simulink model "CRTsfun"  (Simulink 8.0)
settings: Solver=ode45  StartTime=0.0  StopTime=10.0  RelTol=1e-3
undefined symbols (not defined in the file or in its folder): vicrt_initcallback, vicrt_initmexcallback, vicrt_inputfile, vicrt_simulationmanager
(part 2 of 3)

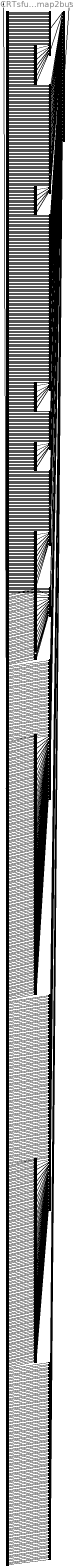
== system CRTsfun/VI-CarRealTime/Output_Bus/IOmap2bus ==
  In : Inport
  Actual_Tread_Speed : BusCreator
  Aggregate_Force_At_Wheel : BusCreator
  Alpha : BusCreator
  Animator_Widget : BusCreator  Inputs=2
  Auxiliary_Roll_Force : BusCreator
  Auxiliary_Roll_Force_at_element : BusCreator  Inputs=2
  Auxiliary_Roll_deformation_at_element : BusCreator  Inputs=2
  Brake : BusCreator  Inputs=7
  Brake_Moment : BusCreator
  Caster_Angle : BusCreator  Inputs=2
  Chamber_Pressure : BusCreator
  Contact_Patch_Global_X : BusCreator
  Contact_Patch_Global_Y : BusCreator
  Contact_Patch_Global_Z : BusCreator
  Contact_Patch_Global_dZdX : BusCreator
  Contact_Patch_Global_dZdY : BusCreator
  Damper : BusCreator  Inputs=5
  Demux : Demux  Outputs=1100
  Drive_Moment : BusCreator
  Effective_Closing_Speed : BusCreator
  Effective_Penetration : BusCreator
  Effective_Rolling_Radius : BusCreator
  Equivalent_Tread_Speed : BusCreator
  Euler_Roll : BusCreator
  External_Friction_Scale_Factor : BusCreator
  Force_At_Bumper : BusCreator
  Force_At_Bumper1 : BusCreator
  Force_At_Damper : BusCreator
  Force_At_Spring : BusCreator
  Force_At_Wheel{,1..3} (4 alike) : BusCreator
  Force_Aux_At_Wheel : BusCreator
  Global_Omega_X : BusCreator
  Global_Omega_Y : BusCreator
  Global_Omega_Z : BusCreator
  Global_Vx : BusCreator
  Global_Vy : BusCreator
  Global_Vz : BusCreator
  Global_X : BusCreator
  Global_Y : BusCreator
  Global_Z : BusCreator
  Ground_Surface_Contact_Patch_Vx : BusCreator
  Ground_Surface_Contact_Patch_Vy : BusCreator
  Ground_Surface_Force_X : BusCreator
  Ground_Surface_Force_Y : BusCreator
  Ground_Surface_Force_Z : BusCreator
  Ground_Surface_Gyroscopic_Moment : BusCreator
  Ground_Surface_Kappa_Fy : BusCreator
  Ground_Surface_Moment_X : BusCreator
  Ground_Surface_Moment_Y : BusCreator
  Ground_Surface_Moment_Z : BusCreator
  Ground_Surface_Peak_Friction_X : BusCreator
  Ground_Surface_Peak_Friction_Y : BusCreator
  Ground_Surface_Residual_Torque : BusCreator
  Ground_Surface_Wheel_Center_Vx : BusCreator
  Gyro : BusCreator  Inputs=10
  Hook_rear : BusCreator  Inputs=18
  Hub_Carrier_Force_Global_X : BusCreator
  Hub_Carrier_Force_Global_Y : BusCreator
  Hub_Carrier_Force_Global_Z : BusCreator
  Hub_Carrier_Force_Local_X : BusCreator
  Hub_Carrier_Force_Local_Y : BusCreator
  Hub_Carrier_Force_Local_Z : BusCreator
  Hub_Carrier_Moment_Global_X : BusCreator
  Hub_Carrier_Moment_Global_Y : BusCreator
  Hub_Carrier_Moment_Global_Z : BusCreator
  Hub_Carrier_Moment_Local_X : BusCreator
  Hub_Carrier_Moment_Local_Y : BusCreator
  Hub_Carrier_Moment_Local_Z : BusCreator
  Hub_Carrier_Omega_X : BusCreator
  Hub_Carrier_Omega_Y : BusCreator
  Hub_Carrier_Omega_Z : BusCreator
  Hub_Carrier_Vx : BusCreator
  Hub_Carrier_Vy : BusCreator
  Hub_Carrier_Vz : BusCreator
  Inclination : BusCreator
  Inst_Stiff_Deflection : BusCreator
  Inst_Stiff_Force : BusCreator
  Jounce{,1..4} (5 alike) : BusCreator
  Jounce_Acceleration{,1..4} (5 alike) : BusCreator
  Jounce_Bumper : BusCreator  Inputs=5
  Jounce_Rate{,1..4} (5 alike) : BusCreator
  Kingpin_Moment : BusCreator  Inputs=1
  Kingpin_Moment1 : BusCreator  Inputs=2
  Lateral_Relaxation_Length : BusCreator
  Lateral_Slip_With_Lag : BusCreator
  Lateral_Slip_Without_Lag : BusCreator
  Loaded_Radius : BusCreator
  Locked_Damper_Moment : BusCreator
  Locked_Moment : BusCreator
  Locked_Spring_Moment : BusCreator
  Locked_Switch : BusCreator
  Lockup_Rotation : BusCreator
  Longitudinal_Relaxation_Length : BusCreator
  Longitudinal_Slip_With_Lag : BusCreator
  Longitudinal_Slip_Without_Lag : BusCreator
  Moment_Arm_Of_Fx : BusCreator
  Omega : BusCreator
  OutputBus : BusCreator  Inputs=92
  PID_CW_At_Spring : BusCreator
  PID_PH_At_Spring : BusCreator
  PID_RH_At_Spring : BusCreator
  Phi : BusCreator
  Pitch : BusCreator
  Pneumatic_Trail : BusCreator
  Psi : BusCreator
  Rebound_Bumper : BusCreator  Inputs=5
  Roll : BusCreator  Inputs=2
  Rotation : BusCreator
  Sensor : BusCreator  Inputs=16
  Side_View_Angle : BusCreator
  Spindle_Steer : BusCreator
  Spring : BusCreator  Inputs=10
  Steering_Instant_Axis_Rotation : BusCreator  Inputs=2
  Steering_System : BusCreator  Inputs=6
  Suspension : BusCreator  Inputs=14
  System : BusCreator
  System_Mass_Center : BusCreator  Inputs=13
  Theta : BusCreator
  TieRod_Force_Left : BusCreator  Inputs=3
  TieRod_Force_Right : BusCreator  Inputs=3
  Tire : BusCreator  Inputs=46
  User_Input_Contact_Patch_Global_Z_Perturbation : BusCreator
  Vehicle : BusCreator  Inputs=46
  Vehicle_States : BusCreator  Inputs=20
  Wheel : BusCreator  Inputs=37
  Yaw : BusCreator
  aero_forces : BusCreator  Inputs=24
  base_acceleration : BusCreator
  base_deformation : BusCreator
  base_velocity : BusCreator
  bul_jounce_stop_data : BusCreator
  bul_rebound_stop_data : BusCreator
  bur_jounce_stop_data : BusCreator
  bur_rebound_stop_data : BusCreator
  bus_dmp_jounce_stop_data : BusCreator  Inputs=6
  bus_ins_jounce_stop_data : BusCreator  Inputs=6
  bus_roll_dmp_jounce_stop_data : BusCreator  Inputs=6
  bus_spr_jounce_stop_data : BusCreator  Inputs=6
  chassis_accelerations : BusCreator  Inputs=6
  chassis_displacements : BusCreator  Inputs=9
  chassis_velocities : BusCreator  Inputs=6
  clutch : BusCreator  Inputs=2
  condition_sensors : BusCreator  Inputs=1
  cp_force_lateralFL : BusCreator  Inputs=3
  cp_force_lateralFR : BusCreator  Inputs=3
  cp_force_lateralRL : BusCreator  Inputs=3
  cp_force_lateralRR : BusCreator  Inputs=3
  cp_force_longitudinalFL : BusCreator  Inputs=3
  cp_force_longitudinalFR : BusCreator  Inputs=3
  cp_force_longitudinalRL : BusCreator  Inputs=3
  cp_force_longitudinalRR : BusCreator  Inputs=3
  cp_force_normalFL : BusCreator  Inputs=3
  cp_force_normalFR : BusCreator  Inputs=3
  cp_force_normalRL : BusCreator  Inputs=3
  cp_force_normalRR : BusCreator  Inputs=3
  cross_weight : BusCreator
  dal_ride_damper_data : BusCreator
  dar_ride_damper_data : BusCreator
  das_ride_damper_data : BusCreator  Inputs=6
  das_roll_damper_data : BusCreator  Inputs=8
  das_third_damper_data : BusCreator  Inputs=6
  differential_speeds : BusCreator  Inputs=6
  differential_torques : BusCreator  Inputs=6
  driver_demands : BusCreator  Inputs=7
  driving_machine_monitor : BusCreator  Inputs=9
  engine : BusCreator  Inputs=7
  fuel_consumption : BusCreator
  ges_chassis_XFORM : BusCreator  Inputs=6
  ges_hub_XFORMFL : BusCreator  Inputs=6
  ges_hub_XFORMFR : BusCreator  Inputs=6
  ges_hub_XFORMRL : BusCreator  Inputs=6
  ges_hub_XFORMRR : BusCreator  Inputs=6
  hub2cp_XFORMFL : BusCreator  Inputs=3
  hub2cp_XFORMFR : BusCreator  Inputs=3
  hub2cp_XFORMRL : BusCreator  Inputs=3
  hub2cp_XFORMRR : BusCreator  Inputs=3
  hub_center_accx : BusCreator
  hub_center_accy : BusCreator
  hub_center_accz : BusCreator
  ins_inerter_data : BusCreator  Inputs=10
  jfs_torsional_stiffness_data : BusCreator  Inputs=12
  nsl_ride_spring_data : BusCreator  Inputs=6
  nsr_ride_spring_data : BusCreator  Inputs=6
  nss_ride_spring_data : BusCreator  Inputs=10
  res_dmp_rebound_stop_data : BusCreator  Inputs=6
  res_ins_rebound_stop_data : BusCreator  Inputs=6
  res_roll_dmp_rebound_stop_data : BusCreator  Inputs=6
  res_spr_rebound_stop_data : BusCreator  Inputs=6
  rhl_front_setup_sensor_data : BusCreator  Inputs=1
  rhr_front_setup_sensor_data : BusCreator  Inputs=1
  rhs_rear_setup_sensor_data : BusCreator  Inputs=1
  til_wheel_tire_forces : BusCreator  Inputs=18
  til_wheel_tire_kinematics : BusCreator  Inputs=9
  til_wheel_tire_rolling_states : BusCreator  Inputs=9
  tir_wheel_tire_forces : BusCreator  Inputs=18
  tir_wheel_tire_kinematics : BusCreator  Inputs=9
  tir_wheel_tire_rolling_states : BusCreator  Inputs=9
  transmission : BusCreator
  ues_third_spring_data : BusCreator  Inputs=6
  upright_accelerometer : BusCreator
  wheel_angles : BusCreator  Inputs=12
  wheel_center_dispx : BusCreator
  wheel_center_dispy : BusCreator
  wheel_center_dispz : BusCreator
  whl_front_wheel_XFORM : BusCreator  Inputs=9
  whl_rear_wheel_XFORM : BusCreator  Inputs=9
  whl_twin_rear_wheel_XFORM : BusCreator  Inputs=9
  whr_front_wheel_XFORM : BusCreator  Inputs=9
  whr_rear_wheel_XFORM : BusCreator  Inputs=9
  whr_twin_rear_wheel_XFORM : BusCreator  Inputs=9
  Out : Outport
  wires:
  Demux/1100 -> cp_force_normalRR/3  "Z"
  Demux/1099 -> cp_force_normalRR/2  "Y"
  Demux/1098 -> cp_force_normalRR/1  "X"
  cp_force_normalRR/1 -> OutputBus/92  "cp_force_normalRR"
  Demux/1097 -> cp_force_lateralRR/3  "Z"
  Demux/1096 -> cp_force_lateralRR/2  "Y"
  Demux/1095 -> cp_force_lateralRR/1  "X"
  cp_force_lateralRR/1 -> OutputBus/91  "cp_force_lateralRR"
  Demux/1094 -> cp_force_longitudinalRR/3  "Z"
  Demux/1093 -> cp_force_longitudinalRR/2  "Y"
  Demux/1092 -> cp_force_longitudinalRR/1  "X"
  cp_force_longitudinalRR/1 -> OutputBus/90  "cp_force_longitudinalRR"
  Demux/1091 -> hub2cp_XFORMRR/3  "Z"
  Demux/1090 -> hub2cp_XFORMRR/2  "Y"
  Demux/1089 -> hub2cp_XFORMRR/1  "X"
  hub2cp_XFORMRR/1 -> OutputBus/89  "hub2cp_XFORMRR"
  Demux/1088 -> ges_hub_XFORMRR/6  "Phi"
  Demux/1087 -> ges_hub_XFORMRR/5  "Theta"
  Demux/1086 -> ges_hub_XFORMRR/4  "Psi"
  Demux/1085 -> ges_hub_XFORMRR/3  "Z"
  Demux/1084 -> ges_hub_XFORMRR/2  "Y"
  Demux/1083 -> ges_hub_XFORMRR/1  "X"
  ges_hub_XFORMRR/1 -> OutputBus/88  "ges_hub_XFORMRR"
  Demux/1082 -> cp_force_normalRL/3  "Z"
  Demux/1081 -> cp_force_normalRL/2  "Y"
  Demux/1080 -> cp_force_normalRL/1  "X"
  cp_force_normalRL/1 -> OutputBus/87  "cp_force_normalRL"
  Demux/1079 -> cp_force_lateralRL/3  "Z"
  Demux/1078 -> cp_force_lateralRL/2  "Y"
  Demux/1077 -> cp_force_lateralRL/1  "X"
  cp_force_lateralRL/1 -> OutputBus/86  "cp_force_lateralRL"
  Demux/1076 -> cp_force_longitudinalRL/3  "Z"
  Demux/1075 -> cp_force_longitudinalRL/2  "Y"
  Demux/1074 -> cp_force_longitudinalRL/1  "X"
  cp_force_longitudinalRL/1 -> OutputBus/85  "cp_force_longitudinalRL"
  Demux/1073 -> hub2cp_XFORMRL/3  "Z"
  Demux/1072 -> hub2cp_XFORMRL/2  "Y"
  Demux/1071 -> hub2cp_XFORMRL/1  "X"
  hub2cp_XFORMRL/1 -> OutputBus/84  "hub2cp_XFORMRL"
  Demux/1070 -> ges_hub_XFORMRL/6  "Phi"
  Demux/1069 -> ges_hub_XFORMRL/5  "Theta"
  Demux/1068 -> ges_hub_XFORMRL/4  "Psi"
  Demux/1067 -> ges_hub_XFORMRL/3  "Z"
  Demux/1066 -> ges_hub_XFORMRL/2  "Y"
  Demux/1065 -> ges_hub_XFORMRL/1  "X"
  ges_hub_XFORMRL/1 -> OutputBus/83  "ges_hub_XFORMRL"
  Demux/1064 -> cp_force_normalFR/3  "Z"
  Demux/1063 -> cp_force_normalFR/2  "Y"
  Demux/1062 -> cp_force_normalFR/1  "X"
  cp_force_normalFR/1 -> OutputBus/82  "cp_force_normalFR"
  Demux/1061 -> cp_force_lateralFR/3  "Z"
  Demux/1060 -> cp_force_lateralFR/2  "Y"
  Demux/1059 -> cp_force_lateralFR/1  "X"
  cp_force_lateralFR/1 -> OutputBus/81  "cp_force_lateralFR"
  Demux/1058 -> cp_force_longitudinalFR/3  "Z"
  Demux/1057 -> cp_force_longitudinalFR/2  "Y"
  Demux/1056 -> cp_force_longitudinalFR/1  "X"
  cp_force_longitudinalFR/1 -> OutputBus/80  "cp_force_longitudinalFR"
  Demux/1055 -> hub2cp_XFORMFR/3  "Z"
  Demux/1054 -> hub2cp_XFORMFR/2  "Y"
  Demux/1053 -> hub2cp_XFORMFR/1  "X"
  hub2cp_XFORMFR/1 -> OutputBus/79  "hub2cp_XFORMFR"
  Demux/1052 -> ges_hub_XFORMFR/6  "Phi"
  Demux/1051 -> ges_hub_XFORMFR/5  "Theta"
  Demux/1050 -> ges_hub_XFORMFR/4  "Psi"
  Demux/1049 -> ges_hub_XFORMFR/3  "Z"
  Demux/1048 -> ges_hub_XFORMFR/2  "Y"
  Demux/1047 -> ges_hub_XFORMFR/1  "X"
  ges_hub_XFORMFR/1 -> OutputBus/78  "ges_hub_XFORMFR"
  Demux/1046 -> cp_force_normalFL/3  "Z"
  Demux/1045 -> cp_force_normalFL/2  "Y"
  Demux/1044 -> cp_force_normalFL/1  "X"
  cp_force_normalFL/1 -> OutputBus/77  "cp_force_normalFL"
  Demux/1043 -> cp_force_lateralFL/3  "Z"
  Demux/1042 -> cp_force_lateralFL/2  "Y"
  Demux/1041 -> cp_force_lateralFL/1  "X"
  cp_force_lateralFL/1 -> OutputBus/76  "cp_force_lateralFL"
  Demux/1040 -> cp_force_longitudinalFL/3  "Z"
  Demux/1039 -> cp_force_longitudinalFL/2  "Y"
  Demux/1038 -> cp_force_longitudinalFL/1  "X"
  cp_force_longitudinalFL/1 -> OutputBus/75  "cp_force_longitudinalFL"
  Demux/1037 -> hub2cp_XFORMFL/3  "Z"
  Demux/1036 -> hub2cp_XFORMFL/2  "Y"
  Demux/1035 -> hub2cp_XFORMFL/1  "X"
  hub2cp_XFORMFL/1 -> OutputBus/74  "hub2cp_XFORMFL"
  Demux/1034 -> ges_hub_XFORMFL/6  "Phi"
  Demux/1033 -> ges_hub_XFORMFL/5  "Theta"
  Demux/1032 -> ges_hub_XFORMFL/4  "Psi"
  Demux/1031 -> ges_hub_XFORMFL/3  "Z"
  Demux/1030 -> ges_hub_XFORMFL/2  "Y"
  Demux/1029 -> ges_hub_XFORMFL/1  "X"
  ges_hub_XFORMFL/1 -> OutputBus/73  "ges_hub_XFORMFL"
  Demux/1028 -> Animator_Widget/2  "engine_rpm"
  Demux/1027 -> Animator_Widget/1  "longitudinal_speed"
  Animator_Widget/1 -> OutputBus/72  "Animator_Widget"
  Demux/1026 -> whr_twin_rear_wheel_XFORM/9  "Z"
  Demux/1025 -> whr_twin_rear_wheel_XFORM/8  "Y"
  Demux/1024 -> whr_twin_rear_wheel_XFORM/7  "X"
  Demux/1023 -> whr_twin_rear_wheel_XFORM/6  "Theta"
  Demux/1022 -> whr_twin_rear_wheel_XFORM/5  "Psi"
  Demux/1021 -> whr_twin_rear_wheel_XFORM/4  "Phi"
  Demux/1020 -> whr_twin_rear_wheel_XFORM/3  "FZ"
  Demux/1019 -> whr_twin_rear_wheel_XFORM/2  "FY"
  Demux/1018 -> whr_twin_rear_wheel_XFORM/1  "FX"
  whr_twin_rear_wheel_XFORM/1 -> OutputBus/71  "whr_twin_rear_wheel_XFORM"
  Demux/1017 -> whr_rear_wheel_XFORM/9  "Z"
  Demux/1016 -> whr_rear_wheel_XFORM/8  "Y"
  Demux/1015 -> whr_rear_wheel_XFORM/7  "X"
  Demux/1014 -> whr_rear_wheel_XFORM/6  "Theta"
  Demux/1013 -> whr_rear_wheel_XFORM/5  "Psi"
  Demux/1012 -> whr_rear_wheel_XFORM/4  "Phi"
  Demux/1011 -> whr_rear_wheel_XFORM/3  "FZ"
  Demux/1010 -> whr_rear_wheel_XFORM/2  "FY"
  Demux/1009 -> whr_rear_wheel_XFORM/1  "FX"
  whr_rear_wheel_XFORM/1 -> OutputBus/70  "whr_rear_wheel_XFORM"
  Demux/1008 -> whr_front_wheel_XFORM/9  "Z"
  Demux/1007 -> whr_front_wheel_XFORM/8  "Y"
  Demux/1006 -> whr_front_wheel_XFORM/7  "X"
  Demux/1005 -> whr_front_wheel_XFORM/6  "Theta"
  Demux/1004 -> whr_front_wheel_XFORM/5  "Psi"
  Demux/1003 -> whr_front_wheel_XFORM/4  "Phi"
  Demux/1002 -> whr_front_wheel_XFORM/3  "FZ"
  Demux/1001 -> whr_front_wheel_XFORM/2  "FY"
  Demux/1000 -> whr_front_wheel_XFORM/1  "FX"
  whr_front_wheel_XFORM/1 -> OutputBus/69  "whr_front_wheel_XFORM"
  Demux/999 -> whl_twin_rear_wheel_XFORM/9  "Z"
  Demux/998 -> whl_twin_rear_wheel_XFORM/8  "Y"
  Demux/997 -> whl_twin_rear_wheel_XFORM/7  "X"
  Demux/996 -> whl_twin_rear_wheel_XFORM/6  "Theta"
  Demux/995 -> whl_twin_rear_wheel_XFORM/5  "Psi"
  Demux/994 -> whl_twin_rear_wheel_XFORM/4  "Phi"
  Demux/993 -> whl_twin_rear_wheel_XFORM/3  "FZ"
  Demux/992 -> whl_twin_rear_wheel_XFORM/2  "FY"
  Demux/991 -> whl_twin_rear_wheel_XFORM/1  "FX"
  whl_twin_rear_wheel_XFORM/1 -> OutputBus/68  "whl_twin_rear_wheel_XFORM"
  Demux/990 -> whl_rear_wheel_XFORM/9  "Z"
  Demux/989 -> whl_rear_wheel_XFORM/8  "Y"
  Demux/988 -> whl_rear_wheel_XFORM/7  "X"
  Demux/987 -> whl_rear_wheel_XFORM/6  "Theta"
  Demux/986 -> whl_rear_wheel_XFORM/5  "Psi"
  Demux/985 -> whl_rear_wheel_XFORM/4  "Phi"
  Demux/984 -> whl_rear_wheel_XFORM/3  "FZ"
  Demux/983 -> whl_rear_wheel_XFORM/2  "FY"
  Demux/982 -> whl_rear_wheel_XFORM/1  "FX"
  whl_rear_wheel_XFORM/1 -> OutputBus/67  "whl_rear_wheel_XFORM"
  Demux/981 -> whl_front_wheel_XFORM/9  "Z"
  Demux/980 -> whl_front_wheel_XFORM/8  "Y"
  Demux/979 -> whl_front_wheel_XFORM/7  "X"
  Demux/978 -> whl_front_wheel_XFORM/6  "Theta"
  Demux/977 -> whl_front_wheel_XFORM/5  "Psi"
  Demux/976 -> whl_front_wheel_XFORM/4  "Phi"
  Demux/975 -> whl_front_wheel_XFORM/3  "FZ"
  Demux/974 -> whl_front_wheel_XFORM/2  "FY"
  Demux/973 -> whl_front_wheel_XFORM/1  "FX"
  whl_front_wheel_XFORM/1 -> OutputBus/66  "whl_front_wheel_XFORM"
  Demux/972 -> wheel_angles/12  "toe_R2"
  Demux/971 -> wheel_angles/11  "toe_R1"
  Demux/970 -> wheel_angles/10  "toe_L2"
  Demux/969 -> wheel_angles/9  "toe_L1"
  Demux/968 -> wheel_angles/8  "caster_R2"
  Demux/967 -> wheel_angles/7  "caster_R1"
  Demux/966 -> wheel_angles/6  "caster_L2"
  Demux/965 -> wheel_angles/5  "caster_L1"
  Demux/964 -> wheel_angles/4  "camber_R2"
  Demux/963 -> wheel_angles/3  "camber_R1"
  Demux/962 -> wheel_angles/2  "camber_L2"
  Demux/961 -> wheel_angles/1  "camber_L1"
  wheel_angles/1 -> OutputBus/65  "wheel_angles"
  Demux/960 -> Yaw/4  "R2"
  Demux/959 -> Yaw/3  "R1"
  Demux/958 -> Yaw/2  "L2"
  Demux/957 -> Yaw/1  "L1"
  Yaw/1 -> Wheel/37  "Yaw"
  Demux/956 -> wheel_center_dispz/4  "rear_right"
  Demux/955 -> wheel_center_dispz/3  "rear_left"
  Demux/954 -> wheel_center_dispz/2  "front_right"
  Demux/953 -> wheel_center_dispz/1  "front_left"
  wheel_center_dispz/1 -> Wheel/36  "wheel_center_dispz"
  Demux/952 -> wheel_center_dispy/4  "rear_right"
  Demux/951 -> wheel_center_dispy/3  "rear_left"
  Demux/950 -> wheel_center_dispy/2  "front_right"
  Demux/949 -> wheel_center_dispy/1  "front_left"
  wheel_center_dispy/1 -> Wheel/35  "wheel_center_dispy"
  Demux/948 -> wheel_center_dispx/4  "rear_right"
  Demux/947 -> wheel_center_dispx/3  "rear_left"
  Demux/946 -> wheel_center_dispx/2  "front_right"
  Demux/945 -> wheel_center_dispx/1  "front_left"
  wheel_center_dispx/1 -> Wheel/34  "wheel_center_dispx"
  Demux/944 -> Theta/4  "R2"
  Demux/943 -> Theta/3  "R1"
  Demux/942 -> Theta/2  "L2"
  Demux/941 -> Theta/1  "L1"
  Theta/1 -> Wheel/33  "Theta"
  Demux/940 -> Spindle_Steer/4  "R2"
  Demux/939 -> Spindle_Steer/3  "R1"
  Demux/938 -> Spindle_Steer/2  "L2"
  Demux/937 -> Spindle_Steer/1  "L1"
  Spindle_Steer/1 -> Wheel/32  "Spindle_Steer"
  Demux/936 -> Side_View_Angle/4  "R2"
  Demux/935 -> Side_View_Angle/3  "R1"
  Demux/934 -> Side_View_Angle/2  "L2"
  Demux/933 -> Side_View_Angle/1  "L1"
  Side_View_Angle/1 -> Wheel/31  "Side_View_Angle"
  Demux/932 -> Rotation/4  "R2"
  Demux/931 -> Rotation/3  "R1"
  Demux/930 -> Rotation/2  "L2"
  Demux/929 -> Rotation/1  "L1"
  Rotation/1 -> Wheel/30  "Rotation"
  Demux/928 -> Psi/4  "R2"
  Demux/927 -> Psi/3  "R1"
  Demux/926 -> Psi/2  "L2"
  Demux/925 -> Psi/1  "L1"
  Psi/1 -> Wheel/29  "Psi"
  Demux/924 -> Pitch/4  "R2"
  Demux/923 -> Pitch/3  "R1"
  Demux/922 -> Pitch/2  "L2"
  Demux/921 -> Pitch/1  "L1"
  Pitch/1 -> Wheel/28  "Pitch"
  Demux/920 -> Phi/4  "R2"
  Demux/919 -> Phi/3  "R1"
  Demux/918 -> Phi/2  "L2"
  Demux/917 -> Phi/1  "L1"
  Phi/1 -> Wheel/27  "Phi"
  Demux/916 -> Omega/4  "R2"
  Demux/915 -> Omega/3  "R1"
  Demux/914 -> Omega/2  "L2"
  Demux/913 -> Omega/1  "L1"
  Omega/1 -> Wheel/26  "Omega"
  Demux/912 -> Kingpin_Moment1/2  "R1"
  Demux/911 -> Kingpin_Moment1/1  "L1"
  Kingpin_Moment1/1 -> Wheel/25  "Kingpin_Moment"
  Demux/910 -> Inclination/4  "R2"
  Demux/909 -> Inclination/3  "R1"
  Demux/908 -> Inclination/2  "L2"
  Demux/907 -> Inclination/1  "L1"
  Inclination/1 -> Wheel/24  "Inclination"
  Demux/906 -> hub_center_accz/4  "rear_right"
  Demux/905 -> hub_center_accz/3  "rear_left"
  Demux/904 -> hub_center_accz/2  "front_right"
  Demux/903 -> hub_center_accz/1  "front_left"
  hub_center_accz/1 -> Wheel/23  "hub_center_accz"
  Demux/902 -> hub_center_accy/4  "rear_right"
  Demux/901 -> hub_center_accy/3  "rear_left"
  Demux/900 -> hub_center_accy/2  "front_right"
  Demux/899 -> hub_center_accy/1  "front_left"
  hub_center_accy/1 -> Wheel/22  "hub_center_accy"
  Demux/898 -> hub_center_accx/4  "rear_right"
  Demux/897 -> hub_center_accx/3  "rear_left"
  Demux/896 -> hub_center_accx/2  "front_right"
  Demux/895 -> hub_center_accx/1  "front_left"
  hub_center_accx/1 -> Wheel/21  "hub_center_accx"
  Demux/894 -> Hub_Carrier_Vz/4  "R2"
  Demux/893 -> Hub_Carrier_Vz/3  "R1"
  Demux/892 -> Hub_Carrier_Vz/2  "L2"
  Demux/891 -> Hub_Carrier_Vz/1  "L1"
  Hub_Carrier_Vz/1 -> Wheel/20  "Hub_Carrier_Vz"
  Demux/890 -> Hub_Carrier_Vy/4  "R2"
  Demux/889 -> Hub_Carrier_Vy/3  "R1"
  Demux/888 -> Hub_Carrier_Vy/2  "L2"
  Demux/887 -> Hub_Carrier_Vy/1  "L1"
  Hub_Carrier_Vy/1 -> Wheel/19  "Hub_Carrier_Vy"
  Demux/886 -> Hub_Carrier_Vx/4  "R2"
  Demux/885 -> Hub_Carrier_Vx/3  "R1"
  Demux/884 -> Hub_Carrier_Vx/2  "L2"
  Demux/883 -> Hub_Carrier_Vx/1  "L1"
  Hub_Carrier_Vx/1 -> Wheel/18  "Hub_Carrier_Vx"
  Demux/882 -> Hub_Carrier_Omega_Z/4  "R2"
  Demux/881 -> Hub_Carrier_Omega_Z/3  "R1"
  Demux/880 -> Hub_Carrier_Omega_Z/2  "L2"
  Demux/879 -> Hub_Carrier_Omega_Z/1  "L1"
  Hub_Carrier_Omega_Z/1 -> Wheel/17  "Hub_Carrier_Omega_Z"
  Demux/878 -> Hub_Carrier_Omega_Y/4  "R2"
  Demux/877 -> Hub_Carrier_Omega_Y/3  "R1"
  Demux/876 -> Hub_Carrier_Omega_Y/2  "L2"
  Demux/875 -> Hub_Carrier_Omega_Y/1  "L1"
  Hub_Carrier_Omega_Y/1 -> Wheel/16  "Hub_Carrier_Omega_Y"
  Demux/874 -> Hub_Carrier_Omega_X/4  "R2"
  Demux/873 -> Hub_Carrier_Omega_X/3  "R1"
  Demux/872 -> Hub_Carrier_Omega_X/2  "L2"
  Demux/871 -> Hub_Carrier_Omega_X/1  "L1"
  Hub_Carrier_Omega_X/1 -> Wheel/15  "Hub_Carrier_Omega_X"
  Demux/870 -> Ground_Surface_Wheel_Center_Vx/4  "R2"
  Demux/869 -> Ground_Surface_Wheel_Center_Vx/3  "R1"
  Demux/868 -> Ground_Surface_Wheel_Center_Vx/2  "L2"
  Demux/867 -> Ground_Surface_Wheel_Center_Vx/1  "L1"
  Ground_Surface_Wheel_Center_Vx/1 -> Wheel/14  "Ground_Surface_Wheel_Center_Vx"
  Demux/866 -> Global_Z/4  "R2"
  Demux/865 -> Global_Z/3  "R1"
  Demux/864 -> Global_Z/2  "L2"
  Demux/863 -> Global_Z/1  "L1"
  Global_Z/1 -> Wheel/13  "Global_Z"
  Demux/862 -> Global_Y/4  "R2"
  Demux/861 -> Global_Y/3  "R1"
  Demux/860 -> Global_Y/2  "L2"
  Demux/859 -> Global_Y/1  "L1"
  Global_Y/1 -> Wheel/12  "Global_Y"
  Demux/858 -> Global_X/4  "R2"
  Demux/857 -> Global_X/3  "R1"
  Demux/856 -> Global_X/2  "L2"
  Demux/855 -> Global_X/1  "L1"
  Global_X/1 -> Wheel/11  "Global_X"
  Demux/854 -> Global_Vz/4  "R2"
  Demux/853 -> Global_Vz/3  "R1"
  Demux/852 -> Global_Vz/2  "L2"
  Demux/851 -> Global_Vz/1  "L1"
  Global_Vz/1 -> Wheel/10  "Global_Vz"
  Demux/850 -> Global_Vy/4  "R2"
  Demux/849 -> Global_Vy/3  "R1"
  Demux/848 -> Global_Vy/2  "L2"
  Demux/847 -> Global_Vy/1  "L1"
  Global_Vy/1 -> Wheel/9  "Global_Vy"
  Demux/846 -> Global_Vx/4  "R2"
  Demux/845 -> Global_Vx/3  "R1"
  Demux/844 -> Global_Vx/2  "L2"
  Demux/843 -> Global_Vx/1  "L1"
  Global_Vx/1 -> Wheel/8  "Global_Vx"
  Demux/842 -> Global_Omega_Z/4  "R2"
  Demux/841 -> Global_Omega_Z/3  "R1"
  Demux/840 -> Global_Omega_Z/2  "L2"
  Demux/839 -> Global_Omega_Z/1  "L1"
  Global_Omega_Z/1 -> Wheel/7  "Global_Omega_Z"
  Demux/838 -> Global_Omega_Y/4  "R2"
  Demux/837 -> Global_Omega_Y/3  "R1"
  Demux/836 -> Global_Omega_Y/2  "L2"
  Demux/835 -> Global_Omega_Y/1  "L1"
  Global_Omega_Y/1 -> Wheel/6  "Global_Omega_Y"
  Demux/834 -> Global_Omega_X/4  "R2"
  Demux/833 -> Global_Omega_X/3  "R1"
  Demux/832 -> Global_Omega_X/2  "L2"
  Demux/831 -> Global_Omega_X/1  "L1"
  Global_Omega_X/1 -> Wheel/5  "Global_Omega_X"
  Demux/830 -> Euler_Roll/4  "R2"
  Demux/829 -> Euler_Roll/3  "R1"
  Demux/828 -> Euler_Roll/2  "L2"
  Demux/827 -> Euler_Roll/1  "L1"
  Euler_Roll/1 -> Wheel/4  "Euler_Roll"
  Demux/826 -> Drive_Moment/4  "R2"
  Demux/825 -> Drive_Moment/3  "R1"
  Demux/824 -> Drive_Moment/2  "L2"
  Demux/823 -> Drive_Moment/1  "L1"
  Drive_Moment/1 -> Wheel/3  "Drive_Moment"
  Demux/822 -> Caster_Angle/2  "right"
  Demux/821 -> Caster_Angle/1  "left"
  Caster_Angle/1 -> Wheel/2  "Caster_Angle"
  Demux/820 -> Alpha/4  "R2"
  Demux/819 -> Alpha/3  "R1"
  Demux/818 -> Alpha/2  "L2"
  Demux/817 -> Alpha/1  "L1"
  Alpha/1 -> Wheel/1  "Alpha"
  Wheel/1 -> OutputBus/64  "Wheel"
  Demux/816 -> Vehicle_States/20  "yaw_angular_vel_wrt_road"
  Demux/815 -> Vehicle_States/19  "yaw_angular_acc_wrt_road"
  Demux/814 -> Vehicle_States/18  "yaw_angle"
  Demux/813 -> Vehicle_States/17  "vertical_vel_wrt_road"
  Demux/812 -> Vehicle_States/16  "vertical_disp"
  Demux/811 -> Vehicle_States/15  "vertical_acc_wrt_road"
  Demux/810 -> Vehicle_States/14  "side_slip"
  Demux/809 -> Vehicle_States/13  "roll_angular_vel_wrt_road"
  Demux/808 -> Vehicle_States/12  "roll_angular_acc_wrt_road"
  Demux/807 -> Vehicle_States/11  "roll_angle"
  Demux/806 -> Vehicle_States/10  "pitch_angular_vel_wrt_road"
  Demux/805 -> Vehicle_States/9  "pitch_angular_acc_wrt_road"
  Demux/804 -> Vehicle_States/8  "pitch_angle"
  Demux/803 -> Vehicle_States/7  "longitudinal_vel_wrt_road"
  Demux/802 -> Vehicle_States/6  "longitudinal_disp"
  Demux/801 -> Vehicle_States/5  "longitudinal_acc_wrt_road"
  Demux/800 -> Vehicle_States/4  "lateral_vel_wrt_road"
  Demux/799 -> Vehicle_States/3  "lateral_disp"
  Demux/798 -> Vehicle_States/2  "lateral_acc_wrt_road"
  Demux/797 -> Vehicle_States/1  "horizontal_vel_wrt_road"
  Vehicle_States/1 -> OutputBus/63  "Vehicle_States"
  Demux/796 -> Vehicle/46  "Yaw"
  Demux/795 -> Vehicle/45  "Understeer_Stability_Factor"
  Demux/794 -> Vehicle/44  "Understeer_Gradient"
  Demux/793 -> Vehicle/43  "Side_Slip_Angle_Rate"
  Demux/792 -> Vehicle/42  "Side_Slip_Angle"
  Demux/791 -> Vehicle/41  "Pitch"
  Demux/790 -> Vehicle/40  "Origin_Global_Z_wrt_road_mk"
  Demux/789 -> Vehicle/39  "Origin_Global_Z"
  Demux/788 -> Vehicle/38  "Origin_Global_Y"
  Demux/787 -> Vehicle/37  "Origin_Global_X"
  Demux/786 -> Vehicle/36  "Origin_Distance_Traveled"
  Demux/785 -> Vehicle/35  "Inclination_Roll"
  Demux/784 -> Vehicle/34  "Global_Omega_Z"
  Demux/783 -> Vehicle/33  "Global_Omega_Y"
  Demux/782 -> Vehicle/32  "Global_Omega_X"
  Demux/781 -> Vehicle/31  "Global_Alpha_Z"
  Demux/780 -> Vehicle/30  "Global_Alpha_Y"
  Demux/779 -> Vehicle/29  "Global_Alpha_X"
  Demux/778 -> Vehicle/28  "front_ride_height_at_center_point"
  Demux/777 -> Vehicle/27  "Euler_Roll"
  Demux/776 -> Vehicle/26  "cross_weight_PID"
  Demux/775 -> Vehicle/25  "CM_Tracking_Vy"
  Demux/774 -> Vehicle/24  "CM_Tracking_Vx"
  Demux/773 -> Vehicle/23  "CM_Tracking_Ay"
  Demux/772 -> Vehicle/22  "CM_Tracking_Ax"
  Demux/771 -> Vehicle/21  "CM_Global_Z"
  Demux/770 -> Vehicle/20  "CM_Global_Y"
  Demux/769 -> Vehicle/19  "CM_Global_X"
  Demux/768 -> Vehicle/18  "CM_Global_Vy"
  Demux/767 -> Vehicle/17  "CM_Global_Vx"
  Demux/766 -> Vehicle/16  "CM_Global_Ay"
  Demux/765 -> Vehicle/15  "CM_Global_Ax"
  Demux/764 -> Vehicle/14  "CM_Global_And_Tracking_Vz"
  Demux/763 -> Vehicle/13  "CM_Global_And_Tracking_Az"
  Demux/762 -> Vehicle/12  "CM_Body_Fixed_Vz"
  Demux/761 -> Vehicle/11  "CM_Body_Fixed_Vy"
  Demux/760 -> Vehicle/10  "CM_Body_Fixed_Vx"
  Demux/759 -> Vehicle/9  "CM_Body_Fixed_Az"
  Demux/758 -> Vehicle/8  "CM_Body_Fixed_Ay"
  Demux/757 -> Vehicle/7  "CM_Body_Fixed_Ax"
  Demux/756 -> Vehicle/6  "Body_Fixed_Omega_Z"
  Demux/755 -> Vehicle/5  "Body_Fixed_Omega_Y"
  Demux/754 -> Vehicle/4  "Body_Fixed_Omega_X"
  Demux/753 -> Vehicle/3  "Body_Fixed_Alpha_Z"
  Demux/752 -> Vehicle/2  "Body_Fixed_Alpha_Y"
  Demux/751 -> Vehicle/1  "Body_Fixed_Alpha_X"
  Vehicle/1 -> OutputBus/62  "Vehicle"
  Demux/750 -> upright_accelerometer/4  "Z_right_rear"
  Demux/749 -> upright_accelerometer/3  "Z_right_front"
  Demux/748 -> upright_accelerometer/2  "Z_left_rear"
  Demux/747 -> upright_accelerometer/1  "Z_left_front"
  upright_accelerometer/1 -> OutputBus/61  "upright_accelerometer"
  Demux/746 -> ues_third_spring_data/6  "velocity_rear"
  Demux/745 -> ues_third_spring_data/5  "velocity_front"
  Demux/744 -> ues_third_spring_data/4  "force_rear"
  Demux/743 -> ues_third_spring_data/3  "force_front"
  Demux/742 -> ues_third_spring_data/2  "displacement_rear"
  Demux/741 -> ues_third_spring_data/1  "displacement_front"
  ues_third_spring_data/1 -> OutputBus/60  "ues_third_spring_data"
  Demux/740 -> transmission/4  "ratio"
  Demux/739 -> transmission/3  "output_rpm"
  Demux/738 -> transmission/2  "input_rpm"
  Demux/737 -> transmission/1  "gear"
  transmission/1 -> OutputBus/59  "transmission"
  Demux/736 -> tir_wheel_tire_rolling_states/9  "rolling_radius_twin_rear"
  Demux/735 -> tir_wheel_tire_rolling_states/8  "rolling_radius_rear"
  Demux/734 -> tir_wheel_tire_rolling_states/7  "rolling_radius_front"
  Demux/733 -> tir_wheel_tire_rolling_states/6  "omega_free_twin_rear"
  Demux/732 -> tir_wheel_tire_rolling_states/5  "omega_free_rear"
  Demux/731 -> tir_wheel_tire_rolling_states/4  "omega_free_front"
  Demux/730 -> tir_wheel_tire_rolling_states/3  "omega_actual_twin_rear"
  Demux/729 -> tir_wheel_tire_rolling_states/2  "omega_actual_rear"
  Demux/728 -> tir_wheel_tire_rolling_states/1  "omega_actual_front"
  tir_wheel_tire_rolling_states/1 -> OutputBus/58  "tir_wheel_tire_rolling_states"
  Demux/727 -> tir_wheel_tire_kinematics/9  "longitudinal_slip_twin_rear"
  Demux/726 -> tir_wheel_tire_kinematics/8  "longitudinal_slip_rear"
  Demux/725 -> tir_wheel_tire_kinematics/7  "longitudinal_slip_front"
  Demux/724 -> tir_wheel_tire_kinematics/6  "lateral_slip_twin_rear"
  Demux/723 -> tir_wheel_tire_kinematics/5  "lateral_slip_rear"
  Demux/722 -> tir_wheel_tire_kinematics/4  "lateral_slip_front"
  Demux/721 -> tir_wheel_tire_kinematics/3  "inclination_angle_twin_rear"
  Demux/720 -> tir_wheel_tire_kinematics/2  "inclination_angle_rear"
  Demux/719 -> tir_wheel_tire_kinematics/1  "inclination_angle_front"
  tir_wheel_tire_kinematics/1 -> OutputBus/57  "tir_wheel_tire_kinematics"
  Demux/718 -> tir_wheel_tire_forces/18  "rolling_resistance_twin_rear"
  Demux/717 -> tir_wheel_tire_forces/17  "rolling_resistance_rear"
  Demux/716 -> tir_wheel_tire_forces/16  "rolling_resistance_front"
  Demux/715 -> tir_wheel_tire_forces/15  "overturning_moment_twin_rear"
  Demux/714 -> tir_wheel_tire_forces/14  "overturning_moment_rear"
  Demux/713 -> tir_wheel_tire_forces/13  "overturning_moment_front"
  Demux/712 -> tir_wheel_tire_forces/12  "normal_twin_rear"
  Demux/711 -> tir_wheel_tire_forces/11  "normal_rear"
  Demux/710 -> tir_wheel_tire_forces/10  "normal_front"
  Demux/709 -> tir_wheel_tire_forces/9  "longitudinal_twin_rear"
  Demux/708 -> tir_wheel_tire_forces/8  "longitudinal_rear"
  Demux/707 -> tir_wheel_tire_forces/7  "longitudinal_front"
  Demux/706 -> tir_wheel_tire_forces/6  "lateral_twin_rear"
  Demux/705 -> tir_wheel_tire_forces/5  "lateral_rear"
  Demux/704 -> tir_wheel_tire_forces/4  "lateral_front"
  Demux/703 -> tir_wheel_tire_forces/3  "aligning_torque_twin_rear"
  Demux/702 -> tir_wheel_tire_forces/2  "aligning_torque_rear"
  Demux/701 -> tir_wheel_tire_forces/1  "aligning_torque_front"
  tir_wheel_tire_forces/1 -> OutputBus/56  "tir_wheel_tire_forces"
  Demux/700 -> User_Input_Contact_Patch_Global_Z_Perturbation/4  "R2"
  Demux/699 -> User_Input_Contact_Patch_Global_Z_Perturbation/3  "R1"
  Demux/698 -> User_Input_Contact_Patch_Global_Z_Perturbation/2  "L2"
  Demux/697 -> User_Input_Contact_Patch_Global_Z_Perturbation/1  "L1"
  User_Input_Contact_Patch_Global_Z_Perturbation/1 -> Tire/46  "User_Input_Contact_Patch_Global_Z_Perturbation"
  Demux/696 -> Pneumatic_Trail/4  "R2"
  Demux/695 -> Pneumatic_Trail/3  "R1"
  Demux/694 -> Pneumatic_Trail/2  "L2"
  Demux/693 -> Pneumatic_Trail/1  "L1"
  Pneumatic_Trail/1 -> Tire/45  "Pneumatic_Trail"
  Demux/692 -> Moment_Arm_Of_Fx/4  "R2"
  Demux/691 -> Moment_Arm_Of_Fx/3  "R1"
  Demux/690 -> Moment_Arm_Of_Fx/2  "L2"
  Demux/689 -> Moment_Arm_Of_Fx/1  "L1"
  Moment_Arm_Of_Fx/1 -> Tire/44  "Moment_Arm_Of_Fx"
  Demux/688 -> Longitudinal_Slip_With_Lag/4  "R2"
  Demux/687 -> Longitudinal_Slip_With_Lag/3  "R1"
  Demux/686 -> Longitudinal_Slip_With_Lag/2  "L2"
  Demux/685 -> Longitudinal_Slip_With_Lag/1  "L1"
  Longitudinal_Slip_With_Lag/1 -> Tire/43  "Longitudinal_Slip_With_Lag"
  Demux/684 -> Longitudinal_Slip_Without_Lag/4  "R2"
  Demux/683 -> Longitudinal_Slip_Without_Lag/3  "R1"
  Demux/682 -> Longitudinal_Slip_Without_Lag/2  "L2"
  Demux/681 -> Longitudinal_Slip_Without_Lag/1  "L1"
  Longitudinal_Slip_Without_Lag/1 -> Tire/42  "Longitudinal_Slip_Without_Lag"
  Demux/680 -> Longitudinal_Relaxation_Length/4  "R2"
  Demux/679 -> Longitudinal_Relaxation_Length/3  "R1"
  Demux/678 -> Longitudinal_Relaxation_Length/2  "L2"
  Demux/677 -> Longitudinal_Relaxation_Length/1  "L1"
  Longitudinal_Relaxation_Length/1 -> Tire/41  "Longitudinal_Relaxation_Length"
  Demux/676 -> Loaded_Radius/4  "R2"
  Demux/675 -> Loaded_Radius/3  "R1"
  Demux/674 -> Loaded_Radius/2  "L2"
  Demux/673 -> Loaded_Radius/1  "L1"
  Loaded_Radius/1 -> Tire/40  "Loaded_Radius"
  Demux/672 -> Lateral_Slip_With_Lag/4  "R2"
  Demux/671 -> Lateral_Slip_With_Lag/3  "R1"
  Demux/670 -> Lateral_Slip_With_Lag/2  "L2"
  Demux/669 -> Lateral_Slip_With_Lag/1  "L1"
  Lateral_Slip_With_Lag/1 -> Tire/39  "Lateral_Slip_With_Lag"
  Demux/668 -> Lateral_Slip_Without_Lag/4  "R2"
  Demux/667 -> Lateral_Slip_Without_Lag/3  "R1"
  Demux/666 -> Lateral_Slip_Without_Lag/2  "L2"
  Demux/665 -> Lateral_Slip_Without_Lag/1  "L1"
  Lateral_Slip_Without_Lag/1 -> Tire/38  "Lateral_Slip_Without_Lag"
  Demux/664 -> Lateral_Relaxation_Length/4  "R2"
  Demux/663 -> Lateral_Relaxation_Length/3  "R1"
  Demux/662 -> Lateral_Relaxation_Length/2  "L2"
  Demux/661 -> Lateral_Relaxation_Length/1  "L1"
  Lateral_Relaxation_Length/1 -> Tire/37  "Lateral_Relaxation_Length"
  Demux/660 -> Hub_Carrier_Moment_Local_Z/4  "R2"
  Demux/659 -> Hub_Carrier_Moment_Local_Z/3  "R1"
  Demux/658 -> Hub_Carrier_Moment_Local_Z/2  "L2"
  Demux/657 -> Hub_Carrier_Moment_Local_Z/1  "L1"
  Hub_Carrier_Moment_Local_Z/1 -> Tire/36  "Hub_Carrier_Moment_Local_Z"
  Demux/656 -> Hub_Carrier_Moment_Local_Y/4  "R2"
  Demux/655 -> Hub_Carrier_Moment_Local_Y/3  "R1"
  Demux/654 -> Hub_Carrier_Moment_Local_Y/2  "L2"
  Demux/653 -> Hub_Carrier_Moment_Local_Y/1  "L1"
  Hub_Carrier_Moment_Local_Y/1 -> Tire/35  "Hub_Carrier_Moment_Local_Y"
  Demux/652 -> Hub_Carrier_Moment_Local_X/4  "R2"
  Demux/651 -> Hub_Carrier_Moment_Local_X/3  "R1"
  Demux/650 -> Hub_Carrier_Moment_Local_X/2  "L2"
  Demux/649 -> Hub_Carrier_Moment_Local_X/1  "L1"
  Hub_Carrier_Moment_Local_X/1 -> Tire/34  "Hub_Carrier_Moment_Local_X"
  Demux/648 -> Hub_Carrier_Moment_Global_Z/4  "R2"
  Demux/647 -> Hub_Carrier_Moment_Global_Z/3  "R1"
  Demux/646 -> Hub_Carrier_Moment_Global_Z/2  "L2"
  Demux/645 -> Hub_Carrier_Moment_Global_Z/1  "L1"
  Hub_Carrier_Moment_Global_Z/1 -> Tire/33  "Hub_Carrier_Moment_Global_Z"
  Demux/644 -> Hub_Carrier_Moment_Global_Y/4  "R2"
  Demux/643 -> Hub_Carrier_Moment_Global_Y/3  "R1"
  Demux/642 -> Hub_Carrier_Moment_Global_Y/2  "L2"
  Demux/641 -> Hub_Carrier_Moment_Global_Y/1  "L1"
  Hub_Carrier_Moment_Global_Y/1 -> Tire/32  "Hub_Carrier_Moment_Global_Y"
  Demux/640 -> Hub_Carrier_Moment_Global_X/4  "R2"
  Demux/639 -> Hub_Carrier_Moment_Global_X/3  "R1"
  Demux/638 -> Hub_Carrier_Moment_Global_X/2  "L2"
  Demux/637 -> Hub_Carrier_Moment_Global_X/1  "L1"
  Hub_Carrier_Moment_Global_X/1 -> Tire/31  "Hub_Carrier_Moment_Global_X"
  Demux/636 -> Hub_Carrier_Force_Local_Z/4  "R2"
  Demux/635 -> Hub_Carrier_Force_Local_Z/3  "R1"
  Demux/634 -> Hub_Carrier_Force_Local_Z/2  "L2"
  Demux/633 -> Hub_Carrier_Force_Local_Z/1  "L1"
  Hub_Carrier_Force_Local_Z/1 -> Tire/30  "Hub_Carrier_Force_Local_Z"
  Demux/632 -> Hub_Carrier_Force_Local_Y/4  "R2"
  Demux/631 -> Hub_Carrier_Force_Local_Y/3  "R1"
  Demux/630 -> Hub_Carrier_Force_Local_Y/2  "L2"
  Demux/629 -> Hub_Carrier_Force_Local_Y/1  "L1"
  Hub_Carrier_Force_Local_Y/1 -> Tire/29  "Hub_Carrier_Force_Local_Y"
  Demux/628 -> Hub_Carrier_Force_Local_X/4  "R2"
  Demux/627 -> Hub_Carrier_Force_Local_X/3  "R1"
  Demux/626 -> Hub_Carrier_Force_Local_X/2  "L2"
  Demux/625 -> Hub_Carrier_Force_Local_X/1  "L1"
  Hub_Carrier_Force_Local_X/1 -> Tire/28  "Hub_Carrier_Force_Local_X"
  Demux/624 -> Hub_Carrier_Force_Global_Z/4  "R2"
  Demux/623 -> Hub_Carrier_Force_Global_Z/3  "R1"
  Demux/622 -> Hub_Carrier_Force_Global_Z/2  "L2"
  Demux/621 -> Hub_Carrier_Force_Global_Z/1  "L1"
  Hub_Carrier_Force_Global_Z/1 -> Tire/27  "Hub_Carrier_Force_Global_Z"
  Demux/620 -> Hub_Carrier_Force_Global_Y/4  "R2"
  Demux/619 -> Hub_Carrier_Force_Global_Y/3  "R1"
  Demux/618 -> Hub_Carrier_Force_Global_Y/2  "L2"
  Demux/617 -> Hub_Carrier_Force_Global_Y/1  "L1"
  Hub_Carrier_Force_Global_Y/1 -> Tire/26  "Hub_Carrier_Force_Global_Y"
  Demux/616 -> Hub_Carrier_Force_Global_X/4  "R2"
  Demux/615 -> Hub_Carrier_Force_Global_X/3  "R1"
  Demux/614 -> Hub_Carrier_Force_Global_X/2  "L2"
  Demux/613 -> Hub_Carrier_Force_Global_X/1  "L1"
  Hub_Carrier_Force_Global_X/1 -> Tire/25  "Hub_Carrier_Force_Global_X"
  Demux/612 -> Ground_Surface_Residual_Torque/4  "R2"
  Demux/611 -> Ground_Surface_Residual_Torque/3  "R1"
  Demux/610 -> Ground_Surface_Residual_Torque/2  "L2"
  Demux/609 -> Ground_Surface_Residual_Torque/1  "L1"
  Ground_Surface_Residual_Torque/1 -> Tire/24  "Ground_Surface_Residual_Torque"
  Demux/608 -> Ground_Surface_Peak_Friction_Y/4  "R2"
  Demux/607 -> Ground_Surface_Peak_Friction_Y/3  "R1"
  Demux/606 -> Ground_Surface_Peak_Friction_Y/2  "L2"
  Demux/605 -> Ground_Surface_Peak_Friction_Y/1  "L1"
  Ground_Surface_Peak_Friction_Y/1 -> Tire/23  "Ground_Surface_Peak_Friction_Y"
  Demux/604 -> Ground_Surface_Peak_Friction_X/4  "R2"
  Demux/603 -> Ground_Surface_Peak_Friction_X/3  "R1"
  Demux/602 -> Ground_Surface_Peak_Friction_X/2  "L2"
  Demux/601 -> Ground_Surface_Peak_Friction_X/1  "L1"
  Ground_Surface_Peak_Friction_X/1 -> Tire/22  "Ground_Surface_Peak_Friction_X"
  Demux/600 -> Ground_Surface_Moment_Z/4  "R2"
  Demux/599 -> Ground_Surface_Moment_Z/3  "R1"
  Demux/598 -> Ground_Surface_Moment_Z/2  "L2"
  Demux/597 -> Ground_Surface_Moment_Z/1  "L1"
  Ground_Surface_Moment_Z/1 -> Tire/21  "Ground_Surface_Moment_Z"
  Demux/596 -> Ground_Surface_Moment_Y/4  "R2"
  Demux/595 -> Ground_Surface_Moment_Y/3  "R1"
  Demux/594 -> Ground_Surface_Moment_Y/2  "L2"
  Demux/593 -> Ground_Surface_Moment_Y/1  "L1"
  Ground_Surface_Moment_Y/1 -> Tire/20  "Ground_Surface_Moment_Y"
  Demux/592 -> Ground_Surface_Moment_X/4  "R2"
  Demux/591 -> Ground_Surface_Moment_X/3  "R1"
  Demux/590 -> Ground_Surface_Moment_X/2  "L2"
  Demux/589 -> Ground_Surface_Moment_X/1  "L1"
  Ground_Surface_Moment_X/1 -> Tire/19  "Ground_Surface_Moment_X"
  Demux/588 -> Ground_Surface_Kappa_Fy/4  "R2"
  Demux/587 -> Ground_Surface_Kappa_Fy/3  "R1"
  Demux/586 -> Ground_Surface_Kappa_Fy/2  "L2"
  Demux/585 -> Ground_Surface_Kappa_Fy/1  "L1"
  Ground_Surface_Kappa_Fy/1 -> Tire/18  "Ground_Surface_Kappa_Fy"
  Demux/584 -> Ground_Surface_Gyroscopic_Moment/4  "R2"
  Demux/583 -> Ground_Surface_Gyroscopic_Moment/3  "R1"
  Demux/582 -> Ground_Surface_Gyroscopic_Moment/2  "L2"
  Demux/581 -> Ground_Surface_Gyroscopic_Moment/1  "L1"
  Ground_Surface_Gyroscopic_Moment/1 -> Tire/17  "Ground_Surface_Gyroscopic_Moment"
  Demux/580 -> Ground_Surface_Force_Z/4  "R2"
  Demux/579 -> Ground_Surface_Force_Z/3  "R1"
  Demux/578 -> Ground_Surface_Force_Z/2  "L2"
  Demux/577 -> Ground_Surface_Force_Z/1  "L1"
  Ground_Surface_Force_Z/1 -> Tire/16  "Ground_Surface_Force_Z"
  Demux/576 -> Ground_Surface_Force_Y/4  "R2"
  Demux/575 -> Ground_Surface_Force_Y/3  "R1"
  Demux/574 -> Ground_Surface_Force_Y/2  "L2"
  Demux/573 -> Ground_Surface_Force_Y/1  "L1"
  Ground_Surface_Force_Y/1 -> Tire/15  "Ground_Surface_Force_Y"
  Demux/572 -> Ground_Surface_Force_X/4  "R2"
  Demux/571 -> Ground_Surface_Force_X/3  "R1"
  Demux/570 -> Ground_Surface_Force_X/2  "L2"
  Demux/569 -> Ground_Surface_Force_X/1  "L1"
  Ground_Surface_Force_X/1 -> Tire/14  "Ground_Surface_Force_X"
  Demux/568 -> Ground_Surface_Contact_Patch_Vy/4  "R2"
  Demux/567 -> Ground_Surface_Contact_Patch_Vy/3  "R1"
  Demux/566 -> Ground_Surface_Contact_Patch_Vy/2  "L2"
  Demux/565 -> Ground_Surface_Contact_Patch_Vy/1  "L1"
  Ground_Surface_Contact_Patch_Vy/1 -> Tire/13  "Ground_Surface_Contact_Patch_Vy"
  Demux/564 -> Ground_Surface_Contact_Patch_Vx/4  "R2"
  Demux/563 -> Ground_Surface_Contact_Patch_Vx/3  "R1"
  Demux/562 -> Ground_Surface_Contact_Patch_Vx/2  "L2"
  Demux/561 -> Ground_Surface_Contact_Patch_Vx/1  "L1"
  Ground_Surface_Contact_Patch_Vx/1 -> Tire/12  "Ground_Surface_Contact_Patch_Vx"
  Demux/560 -> External_Friction_Scale_Factor/4  "R2"
  Demux/559 -> External_Friction_Scale_Factor/3  "R1"
  Demux/558 -> External_Friction_Scale_Factor/2  "L2"
  Demux/557 -> External_Friction_Scale_Factor/1  "L1"
  External_Friction_Scale_Factor/1 -> Tire/11  "External_Friction_Scale_Factor"
  Demux/556 -> Equivalent_Tread_Speed/4  "R2"
  Demux/555 -> Equivalent_Tread_Speed/3  "R1"
  Demux/554 -> Equivalent_Tread_Speed/2  "L2"
  Demux/553 -> Equivalent_Tread_Speed/1  "L1"
  Equivalent_Tread_Speed/1 -> Tire/10  "Equivalent_Tread_Speed"
  Demux/552 -> Effective_Rolling_Radius/4  "R2"
  Demux/551 -> Effective_Rolling_Radius/3  "R1"
  Demux/550 -> Effective_Rolling_Radius/2  "L2"
  Demux/549 -> Effective_Rolling_Radius/1  "L1"
  Effective_Rolling_Radius/1 -> Tire/9  "Effective_Rolling_Radius"
  Demux/548 -> Effective_Penetration/4  "R2"
  Demux/547 -> Effective_Penetration/3  "R1"
  Demux/546 -> Effective_Penetration/2  "L2"
  Demux/545 -> Effective_Penetration/1  "L1"
  Effective_Penetration/1 -> Tire/8  "Effective_Penetration"
  Demux/544 -> Effective_Closing_Speed/4  "R2"
  Demux/543 -> Effective_Closing_Speed/3  "R1"
  Demux/542 -> Effective_Closing_Speed/2  "L2"
  Demux/541 -> Effective_Closing_Speed/1  "L1"
  Effective_Closing_Speed/1 -> Tire/7  "Effective_Closing_Speed"
  Demux/540 -> Contact_Patch_Global_Z/4  "R2"
  Demux/539 -> Contact_Patch_Global_Z/3  "R1"
  Demux/538 -> Contact_Patch_Global_Z/2  "L2"
  Demux/537 -> Contact_Patch_Global_Z/1  "L1"
  Contact_Patch_Global_Z/1 -> Tire/6  "Contact_Patch_Global_Z"
  Demux/536 -> Contact_Patch_Global_Y/4  "R2"
  Demux/535 -> Contact_Patch_Global_Y/3  "R1"
  Demux/534 -> Contact_Patch_Global_Y/2  "L2"
  Demux/533 -> Contact_Patch_Global_Y/1  "L1"
  Contact_Patch_Global_Y/1 -> Tire/5  "Contact_Patch_Global_Y"
  Demux/532 -> Contact_Patch_Global_X/4  "R2"
  Demux/531 -> Contact_Patch_Global_X/3  "R1"
  Demux/530 -> Contact_Patch_Global_X/2  "L2"
  Demux/529 -> Contact_Patch_Global_X/1  "L1"
  Contact_Patch_Global_X/1 -> Tire/4  "Contact_Patch_Global_X"
  Demux/528 -> Contact_Patch_Global_dZdY/4  "R2"
  Demux/527 -> Contact_Patch_Global_dZdY/3  "R1"
  Demux/526 -> Contact_Patch_Global_dZdY/2  "L2"
  Demux/525 -> Contact_Patch_Global_dZdY/1  "L1"
  Contact_Patch_Global_dZdY/1 -> Tire/3  "Contact_Patch_Global_dZdY"
  Demux/524 -> Contact_Patch_Global_dZdX/4  "R2"
  Demux/523 -> Contact_Patch_Global_dZdX/3  "R1"
  Demux/522 -> Contact_Patch_Global_dZdX/2  "L2"
  Demux/521 -> Contact_Patch_Global_dZdX/1  "L1"
  Contact_Patch_Global_dZdX/1 -> Tire/2  "Contact_Patch_Global_dZdX"
  Demux/520 -> Actual_Tread_Speed/4  "R2"
  Demux/519 -> Actual_Tread_Speed/3  "R1"
  Demux/518 -> Actual_Tread_Speed/2  "L2"
  Demux/517 -> Actual_Tread_Speed/1  "L1"
  Actual_Tread_Speed/1 -> Tire/1  "Actual_Tread_Speed"
  Tire/1 -> OutputBus/55  "Tire"
  Demux/516 -> til_wheel_tire_rolling_states/9  "rolling_radius_twin_rear"
  Demux/515 -> til_wheel_tire_rolling_states/8  "rolling_radius_rear"
  Demux/514 -> til_wheel_tire_rolling_states/7  "rolling_radius_front"
  Demux/513 -> til_wheel_tire_rolling_states/6  "omega_free_twin_rear"
  Demux/512 -> til_wheel_tire_rolling_states/5  "omega_free_rear"
  Demux/511 -> til_wheel_tire_rolling_states/4  "omega_free_front"
  Demux/510 -> til_wheel_tire_rolling_states/3  "omega_actual_twin_rear"
  Demux/509 -> til_wheel_tire_rolling_states/2  "omega_actual_rear"
  Demux/508 -> til_wheel_tire_rolling_states/1  "omega_actual_front"
  til_wheel_tire_rolling_states/1 -> OutputBus/54  "til_wheel_tire_rolling_states"
  Demux/507 -> til_wheel_tire_kinematics/9  "longitudinal_slip_twin_rear"
  Demux/506 -> til_wheel_tire_kinematics/8  "longitudinal_slip_rear"
  Demux/505 -> til_wheel_tire_kinematics/7  "longitudinal_slip_front"
  Demux/504 -> til_wheel_tire_kinematics/6  "lateral_slip_twin_rear"
  Demux/503 -> til_wheel_tire_kinematics/5  "lateral_slip_rear"
  Demux/502 -> til_wheel_tire_kinematics/4  "lateral_slip_front"
  Demux/501 -> til_wheel_tire_kinematics/3  "inclination_angle_twin_rear"
  Demux/500 -> til_wheel_tire_kinematics/2  "inclination_angle_rear"
  Demux/499 -> til_wheel_tire_kinematics/1  "inclination_angle_front"
  til_wheel_tire_kinematics/1 -> OutputBus/53  "til_wheel_tire_kinematics"
  Demux/498 -> til_wheel_tire_forces/18  "rolling_resistance_twin_rear"
  Demux/497 -> til_wheel_tire_forces/17  "rolling_resistance_rear"
  Demux/496 -> til_wheel_tire_forces/16  "rolling_resistance_front"
  Demux/495 -> til_wheel_tire_forces/15  "overturning_moment_twin_rear"
  Demux/494 -> til_wheel_tire_forces/14  "overturning_moment_rear"
  Demux/493 -> til_wheel_tire_forces/13  "overturning_moment_front"
  Demux/492 -> til_wheel_tire_forces/12  "normal_twin_rear"
  Demux/491 -> til_wheel_tire_forces/11  "normal_rear"
  Demux/490 -> til_wheel_tire_forces/10  "normal_front"
  Demux/489 -> til_wheel_tire_forces/9  "longitudinal_twin_rear"
  Demux/488 -> til_wheel_tire_forces/8  "longitudinal_rear"
  Demux/487 -> til_wheel_tire_forces/7  "longitudinal_front"
  Demux/486 -> til_wheel_tire_forces/6  "lateral_twin_rear"
  Demux/485 -> til_wheel_tire_forces/5  "lateral_rear"
  Demux/484 -> til_wheel_tire_forces/4  "lateral_front"
  Demux/483 -> til_wheel_tire_forces/3  "aligning_torque_twin_rear"
  Demux/482 -> til_wheel_tire_forces/2  "aligning_torque_rear"
  Demux/481 -> til_wheel_tire_forces/1  "aligning_torque_front"
  til_wheel_tire_forces/1 -> OutputBus/52  "til_wheel_tire_forces"
  Demux/480 -> System_Mass_Center/13  "Tangential_Acceleration"
  Demux/479 -> System_Mass_Center/12  "Speed"
  Demux/478 -> System_Mass_Center/11  "Path_Curvature"
  Demux/477 -> System_Mass_Center/10  "Normal_Acceleration"
  Demux/476 -> System_Mass_Center/9  "Global_Z"
  Demux/475 -> System_Mass_Center/8  "Global_Y"
  Demux/474 -> System_Mass_Center/7  "Global_X"
  Demux/473 -> System_Mass_Center/6  "Global_Vz"
  Demux/472 -> System_Mass_Center/5  "Global_Vy"
  Demux/471 -> System_Mass_Center/4  "Global_Vx"
  Demux/470 -> System_Mass_Center/3  "Global_Az"
  Demux/469 -> System_Mass_Center/2  "Global_Ay"
  Demux/468 -> System_Mass_Center/1  "Global_Ax"
  System_Mass_Center/1 -> OutputBus/51  "System_Mass_Center"
  Demux/467 -> System/4  "Translational_Speed_Norm"
  Demux/466 -> System/3  "Translational_Acceleration_Norm"
  Demux/465 -> System/2  "Angular_Speed_Norm"
  Demux/464 -> System/1  "Angular_Acceleration_Norm"
  System/1 -> OutputBus/50  "System"
  Demux/463 -> Steering_Instant_Axis_Rotation/2  "R1"
  Demux/462 -> Steering_Instant_Axis_Rotation/1  "L1"
  Steering_Instant_Axis_Rotation/1 -> Suspension/14  "Steering_Instant_Axis_Rotation"
  Demux/461 -> Roll/2  "SUSP2"
  Demux/460 -> Roll/1  "SUSP1"
  Roll/1 -> Suspension/13  "Roll"
  Demux/459 -> Kingpin_Moment/1  "SUSP1"
  Kingpin_Moment/1 -> Suspension/12  "Kingpin_Moment"
  Demux/458 -> Jounce_Rate4/4  "R2"
  Demux/457 -> Jounce_Rate4/3  "R1"
  Demux/456 -> Jounce_Rate4/2  "L2"
  Demux/455 -> Jounce_Rate4/1  "L1"
  Jounce_Rate4/1 -> Suspension/11  "Jounce_Rate"
  Demux/454 -> Jounce_Acceleration4/4  "R2"
  Demux/453 -> Jounce_Acceleration4/3  "R1"
  Demux/452 -> Jounce_Acceleration4/2  "L2"
  Demux/451 -> Jounce_Acceleration4/1  "L1"
  Jounce_Acceleration4/1 -> Suspension/10  "Jounce_Acceleration"
  Demux/450 -> Jounce4/4  "R2"
  Demux/449 -> Jounce4/3  "R1"
  Demux/448 -> Jounce4/2  "L2"
  Demux/447 -> Jounce4/1  "L1"
  Jounce4/1 -> Suspension/9  "Jounce"
  Demux/446 -> Inst_Stiff_Force/4  "rear_right"
  Demux/445 -> Inst_Stiff_Force/3  "rear_left"
  Demux/444 -> Inst_Stiff_Force/2  "front_right"
  Demux/443 -> Inst_Stiff_Force/1  "front_left"
  Inst_Stiff_Force/1 -> Suspension/8  "Inst_Stiff_Force"
  Demux/442 -> Inst_Stiff_Deflection/4  "rear_right"
  Demux/441 -> Inst_Stiff_Deflection/3  "rear_left"
  Demux/440 -> Inst_Stiff_Deflection/2  "front_right"
  Demux/439 -> Inst_Stiff_Deflection/1  "front_left"
  Inst_Stiff_Deflection/1 -> Suspension/7  "Inst_Stiff_Deflection"
  Demux/438 -> base_velocity/4  "R2"
  Demux/437 -> base_velocity/3  "R1"
  Demux/436 -> base_velocity/2  "L2"
  Demux/435 -> base_velocity/1  "L1"
  base_velocity/1 -> Suspension/6  "base_velocity"
  Demux/434 -> base_deformation/4  "R2"
  Demux/433 -> base_deformation/3  "R1"
  Demux/432 -> base_deformation/2  "L2"
  Demux/431 -> base_deformation/1  "L1"
  base_deformation/1 -> Suspension/5  "base_deformation"
  Demux/430 -> base_acceleration/4  "R2"
  Demux/429 -> base_acceleration/3  "R1"
  Demux/428 -> base_acceleration/2  "L2"
  Demux/427 -> base_acceleration/1  "L1"
  base_acceleration/1 -> Suspension/4  "base_acceleration"
  Demux/426 -> Auxiliary_Roll_Force_at_element/2  "SUSP2"
  Demux/425 -> Auxiliary_Roll_Force_at_element/1  "SUSP1"
  Auxiliary_Roll_Force_at_element/1 -> Suspension/3  "Auxiliary_Roll_Force_at_element"
  Demux/424 -> Auxiliary_Roll_Force/4  "SUSP_R2"
  Demux/423 -> Auxiliary_Roll_Force/3  "SUSP_R1"
  Demux/422 -> Auxiliary_Roll_Force/2  "SUSP_L2"
  Demux/421 -> Auxiliary_Roll_Force/1  "SUSP_L1"
  Auxiliary_Roll_Force/1 -> Suspension/2  "Auxiliary_Roll_Force"
  Demux/420 -> Auxiliary_Roll_deformation_at_element/2  "SUSP2"
  Demux/419 -> Auxiliary_Roll_deformation_at_element/1  "SUSP1"
  Auxiliary_Roll_deformation_at_element/1 -> Suspension/1  "Auxiliary_Roll_deformation_at_element"
  Suspension/1 -> OutputBus/49  "Suspension"
  Demux/418 -> TieRod_Force_Right/3  "Z"
  Demux/417 -> TieRod_Force_Right/2  "Y"
  Demux/416 -> TieRod_Force_Right/1  "X"
  TieRod_Force_Right/1 -> Steering_System/6  "TieRod_Force_Right"
  Demux/415 -> TieRod_Force_Left/3  "Z"
  Demux/414 -> TieRod_Force_Left/2  "Y"
  Demux/413 -> TieRod_Force_Left/1  "X"
  TieRod_Force_Left/1 -> Steering_System/5  "TieRod_Force_Left"
  Demux/412 -> Steering_System/4  "Steering_Wheel_Torque"
  Demux/411 -> Steering_System/3  "Steering_column_deformation"
  Demux/410 -> Steering_System/2  "Rack_Force"
  Demux/409 -> Steering_System/1  "Rack_displacement"
  Steering_System/1 -> OutputBus/48  "Steering_System"
  Demux/408 -> PID_RH_At_Spring/4  "R2"
  Demux/407 -> PID_RH_At_Spring/3  "R1"
  Demux/406 -> PID_RH_At_Spring/2  "L2"
  Demux/405 -> PID_RH_At_Spring/1  "L1"
  PID_RH_At_Spring/1 -> Spring/10  "PID_RH_At_Spring"
  Demux/404 -> PID_PH_At_Spring/4  "R2"
  Demux/403 -> PID_PH_At_Spring/3  "R1"
  Demux/402 -> PID_PH_At_Spring/2  "L2"
  Demux/401 -> PID_PH_At_Spring/1  "L1"
  PID_PH_At_Spring/1 -> Spring/9  "PID_PH_At_Spring"
  Demux/400 -> PID_CW_At_Spring/4  "R2"
  Demux/399 -> PID_CW_At_Spring/3  "R1"
  Demux/398 -> PID_CW_At_Spring/2  "L2"
  Demux/397 -> PID_CW_At_Spring/1  "L1"
  PID_CW_At_Spring/1 -> Spring/8  "PID_CW_At_Spring"
  Demux/396 -> Jounce_Rate3/4  "R2"
  Demux/395 -> Jounce_Rate3/3  "R1"
  Demux/394 -> Jounce_Rate3/2  "L2"
  Demux/393 -> Jounce_Rate3/1  "L1"
  Jounce_Rate3/1 -> Spring/7  "Jounce_Rate"
  Demux/392 -> Jounce_Acceleration3/4  "R2"
  Demux/391 -> Jounce_Acceleration3/3  "R1"
  Demux/390 -> Jounce_Acceleration3/2  "L2"
  Demux/389 -> Jounce_Acceleration3/1  "L1"
  Jounce_Acceleration3/1 -> Spring/6  "Jounce_Acceleration"
  Demux/388 -> Jounce3/4  "R2"
  Demux/387 -> Jounce3/3  "R1"
  Demux/386 -> Jounce3/2  "L2"
  Demux/385 -> Jounce3/1  "L1"
  Jounce3/1 -> Spring/5  "Jounce"
  Demux/384 -> Force_Aux_At_Wheel/4  "R2"
  Demux/383 -> Force_Aux_At_Wheel/3  "R1"
  Demux/382 -> Force_Aux_At_Wheel/2  "L2"
  Demux/381 -> Force_Aux_At_Wheel/1  "L1"
  Force_Aux_At_Wheel/1 -> Spring/4  "Force_Aux_At_Wheel"
  Demux/380 -> Force_At_Wheel3/4  "R2"
  Demux/379 -> Force_At_Wheel3/3  "R1"
  Demux/378 -> Force_At_Wheel3/2  "L2"
  Demux/377 -> Force_At_Wheel3/1  "L1"
  Force_At_Wheel3/1 -> Spring/3  "Force_At_Wheel"
  Demux/376 -> Force_At_Spring/4  "R2"
  Demux/375 -> Force_At_Spring/3  "R1"
  Demux/374 -> Force_At_Spring/2  "L2"
  Demux/373 -> Force_At_Spring/1  "L1"
  Force_At_Spring/1 -> Spring/2  "Force_At_Spring"
  Demux/372 -> Aggregate_Force_At_Wheel/4  "R2"
  Demux/371 -> Aggregate_Force_At_Wheel/3  "R1"
  Demux/370 -> Aggregate_Force_At_Wheel/2  "L2"
  Demux/369 -> Aggregate_Force_At_Wheel/1  "L1"
  Aggregate_Force_At_Wheel/1 -> Spring/1  "Aggregate_Force_At_Wheel"
  Spring/1 -> OutputBus/47  "Spring"
  Demux/368 -> Sensor/16  "YawRate_gyro"
  Demux/367 -> Sensor/15  "Vz"
  Demux/366 -> Sensor/14  "Vy"
  Demux/365 -> Sensor/13  "Vx_gyro"
  Demux/364 -> Sensor/12  "Vx"
  Demux/363 -> Sensor/11  "Global_Z"
  Demux/362 -> Sensor/10  "Global_Y"
  Demux/361 -> Sensor/9  "Global_X"
  Demux/360 -> Sensor/8  "Az_Without_Gravity"
  Demux/359 -> Sensor/7  "Az"
  Demux/358 -> Sensor/6  "Ay_Without_Gravity"
  Demux/357 -> Sensor/5  "Ay"
  Demux/356 -> Sensor/4  "Ax_Without_Gravity"
  Demux/355 -> Sensor/3  "Ax"
  Demux/354 -> Sensor/2  "AccY_gyro"
  Demux/353 -> Sensor/1  "AccX_gyro"
  Sensor/1 -> OutputBus/46  "Sensor"
  Demux/352 -> rhs_rear_setup_sensor_data/1  "ride_height"
  rhs_rear_setup_sensor_data/1 -> OutputBus/45  "rhs_rear_setup_sensor_data"
  Demux/351 -> rhr_front_setup_sensor_data/1  "ride_height"
  rhr_front_setup_sensor_data/1 -> OutputBus/44  "rhr_front_setup_sensor_data"
  Demux/350 -> rhl_front_setup_sensor_data/1  "ride_height"
  rhl_front_setup_sensor_data/1 -> OutputBus/43  "rhl_front_setup_sensor_data"
  Demux/349 -> res_spr_rebound_stop_data/6  "velocity_rear"
  Demux/348 -> res_spr_rebound_stop_data/5  "velocity_front"
  Demux/347 -> res_spr_rebound_stop_data/4  "force_rear"
  Demux/346 -> res_spr_rebound_stop_data/3  "force_front"
  Demux/345 -> res_spr_rebound_stop_data/2  "displacement_rear"
  Demux/344 -> res_spr_rebound_stop_data/1  "displacement_front"
  res_spr_rebound_stop_data/1 -> OutputBus/42  "res_spr_rebound_stop_data"
  Demux/343 -> res_roll_dmp_rebound_stop_data/6  "velocity_rear"
  Demux/342 -> res_roll_dmp_rebound_stop_data/5  "velocity_front"
  Demux/341 -> res_roll_dmp_rebound_stop_data/4  "force_rear"
  Demux/340 -> res_roll_dmp_rebound_stop_data/3  "force_front"
  Demux/339 -> res_roll_dmp_rebound_stop_data/2  "displacement_rear"
  Demux/338 -> res_roll_dmp_rebound_stop_data/1  "displacement_front"
  res_roll_dmp_rebound_stop_data/1 -> OutputBus/41  "res_roll_dmp_rebound_stop_data"
  Demux/337 -> res_ins_rebound_stop_data/6  "velocity_rear"
  Demux/336 -> res_ins_rebound_stop_data/5  "velocity_front"
  Demux/335 -> res_ins_rebound_stop_data/4  "force_rear"
  Demux/334 -> res_ins_rebound_stop_data/3  "force_front"
  Demux/333 -> res_ins_rebound_stop_data/2  "displacement_rear"
  Demux/332 -> res_ins_rebound_stop_data/1  "displacement_front"
  res_ins_rebound_stop_data/1 -> OutputBus/40  "res_ins_rebound_stop_data"
  Demux/331 -> res_dmp_rebound_stop_data/6  "velocity_rear"
  Demux/330 -> res_dmp_rebound_stop_data/5  "velocity_front"
  Demux/329 -> res_dmp_rebound_stop_data/4  "force_rear"
  Demux/328 -> res_dmp_rebound_stop_data/3  "force_front"
  Demux/327 -> res_dmp_rebound_stop_data/2  "displacement_rear"
  Demux/326 -> res_dmp_rebound_stop_data/1  "displacement_front"
  res_dmp_rebound_stop_data/1 -> OutputBus/39  "res_dmp_rebound_stop_data"
  Demux/325 -> Jounce_Rate2/4  "R2"
  Demux/324 -> Jounce_Rate2/3  "R1"
  Demux/323 -> Jounce_Rate2/2  "L2"
  Demux/322 -> Jounce_Rate2/1  "L1"
  Jounce_Rate2/1 -> Rebound_Bumper/5  "Jounce_Rate"
  Demux/321 -> Jounce_Acceleration2/4  "R2"
  Demux/320 -> Jounce_Acceleration2/3  "R1"
  Demux/319 -> Jounce_Acceleration2/2  "L2"
  Demux/318 -> Jounce_Acceleration2/1  "L1"
  Jounce_Acceleration2/1 -> Rebound_Bumper/4  "Jounce_Acceleration"
  Demux/317 -> Jounce2/4  "R2"
  Demux/316 -> Jounce2/3  "R1"
  Demux/315 -> Jounce2/2  "L2"
  Demux/314 -> Jounce2/1  "L1"
  Jounce2/1 -> Rebound_Bumper/3  "Jounce"
  Demux/313 -> Force_At_Wheel2/4  "R2"
  Demux/312 -> Force_At_Wheel2/3  "R1"
  Demux/311 -> Force_At_Wheel2/2  "L2"
  Demux/310 -> Force_At_Wheel2/1  "L1"
  Force_At_Wheel2/1 -> Rebound_Bumper/2  "Force_At_Wheel"
  Demux/309 -> Force_At_Bumper1/4  "R2"
  Demux/308 -> Force_At_Bumper1/3  "R1"
  Demux/307 -> Force_At_Bumper1/2  "L2"
  Demux/306 -> Force_At_Bumper1/1  "L1"
  Force_At_Bumper1/1 -> Rebound_Bumper/1  "Force_At_Bumper"
  Rebound_Bumper/1 -> OutputBus/38  "Rebound_Bumper"
  Demux/305 -> nss_ride_spring_data/10  "velocity_rear"
  Demux/304 -> nss_ride_spring_data/9  "velocity_front"
  Demux/303 -> nss_ride_spring_data/8  "PID_PH_At_Spring_rear"
  Demux/302 -> nss_ride_spring_data/7  "PID_PH_At_Spring_front"
  Demux/301 -> nss_ride_spring_data/6  "force_rear"
  Demux/300 -> nss_ride_spring_data/5  "force_front"
  Demux/299 -> nss_ride_spring_data/4  "force_at_wheel_rear"
  Demux/298 -> nss_ride_spring_data/3  "force_at_wheel_front"
  Demux/297 -> nss_ride_spring_data/2  "displacement_rear"
  Demux/296 -> nss_ride_spring_data/1  "displacement_front"
  nss_ride_spring_data/1 -> OutputBus/37  "nss_ride_spring_data"
  Demux/295 -> nsr_ride_spring_data/6  "velocity_rear"
  Demux/294 -> nsr_ride_spring_data/5  "velocity_front"
  Demux/293 -> nsr_ride_spring_data/4  "force_rear"
  Demux/292 -> nsr_ride_spring_data/3  "force_front"
  Demux/291 -> nsr_ride_spring_data/2  "displacement_rear"
  Demux/290 -> nsr_ride_spring_data/1  "displacement_front"
  nsr_ride_spring_data/1 -> OutputBus/36  "nsr_ride_spring_data"
  Demux/289 -> nsl_ride_spring_data/6  "velocity_rear"
  Demux/288 -> nsl_ride_spring_data/5  "velocity_front"
  Demux/287 -> nsl_ride_spring_data/4  "force_rear"
  Demux/286 -> nsl_ride_spring_data/3  "force_front"
  Demux/285 -> nsl_ride_spring_data/2  "displacement_rear"
  Demux/284 -> nsl_ride_spring_data/1  "displacement_front"
  nsl_ride_spring_data/1 -> OutputBus/35  "nsl_ride_spring_data"
  Demux/283 -> Jounce_Rate1/4  "R2"
  Demux/282 -> Jounce_Rate1/3  "R1"
  Demux/281 -> Jounce_Rate1/2  "L2"
  Demux/280 -> Jounce_Rate1/1  "L1"
  Jounce_Rate1/1 -> Jounce_Bumper/5  "Jounce_Rate"
  Demux/279 -> Jounce_Acceleration1/4  "R2"
  Demux/278 -> Jounce_Acceleration1/3  "R1"
  Demux/277 -> Jounce_Acceleration1/2  "L2"
  Demux/276 -> Jounce_Acceleration1/1  "L1"
  Jounce_Acceleration1/1 -> Jounce_Bumper/4  "Jounce_Acceleration"
  Demux/275 -> Jounce1/4  "R2"
  Demux/274 -> Jounce1/3  "R1"
  Demux/273 -> Jounce1/2  "L2"
  Demux/272 -> Jounce1/1  "L1"
  Jounce1/1 -> Jounce_Bumper/3  "Jounce"
  Demux/271 -> Force_At_Wheel1/4  "R2"
  Demux/270 -> Force_At_Wheel1/3  "R1"
  Demux/269 -> Force_At_Wheel1/2  "L2"
  Demux/268 -> Force_At_Wheel1/1  "L1"
  Force_At_Wheel1/1 -> Jounce_Bumper/2  "Force_At_Wheel"
  Demux/267 -> Force_At_Bumper/4  "R2"
  Demux/266 -> Force_At_Bumper/3  "R1"
  Demux/265 -> Force_At_Bumper/2  "L2"
  Demux/264 -> Force_At_Bumper/1  "L1"
  Force_At_Bumper/1 -> Jounce_Bumper/1  "Force_At_Bumper"
  Jounce_Bumper/1 -> OutputBus/34  "Jounce_Bumper"
  Demux/263 -> jfs_torsional_stiffness_data/12  "Z_1"
  Demux/262 -> jfs_torsional_stiffness_data/11  "Y_1"
  Demux/261 -> jfs_torsional_stiffness_data/10  "X_1"
  Demux/260 -> jfs_torsional_stiffness_data/9  "TZ_1"
  Demux/259 -> jfs_torsional_stiffness_data/8  "TY_1"
  Demux/258 -> jfs_torsional_stiffness_data/7  "TX_1"
  Demux/257 -> jfs_torsional_stiffness_data/6  "FZ_1"
  Demux/256 -> jfs_torsional_stiffness_data/5  "FY_1"
  Demux/255 -> jfs_torsional_stiffness_data/4  "FX_1"
  Demux/254 -> jfs_torsional_stiffness_data/3  "AZ_1"
  Demux/253 -> jfs_torsional_stiffness_data/2  "AY_1"
  Demux/252 -> jfs_torsional_stiffness_data/1  "AX_1"
  jfs_torsional_stiffness_data/1 -> OutputBus/33  "jfs_torsional_stiffness_data"
  Demux/251 -> ins_inerter_data/10  "velocity_rear"
  Demux/250 -> ins_inerter_data/9  "velocity_front"
  Demux/249 -> ins_inerter_data/8  "force_rear"
  Demux/248 -> ins_inerter_data/7  "force_front"
  Demux/247 -> ins_inerter_data/6  "force_at_wheel_rear"
  Demux/246 -> ins_inerter_data/5  "force_at_wheel_front"
  Demux/245 -> ins_inerter_data/4  "displacement_rear"
  Demux/244 -> ins_inerter_data/3  "displacement_front"
  Demux/243 -> ins_inerter_data/2  "acceleration_rear"
  Demux/242 -> ins_inerter_data/1  "acceleration_front"
  ins_inerter_data/1 -> OutputBus/32  "ins_inerter_data"
  Demux/241 -> Hook_rear/18  "Local_Moment_Z"
  Demux/240 -> Hook_rear/17  "Local_Moment_Y"
  Demux/239 -> Hook_rear/16  "Local_Moment_X"
  Demux/238 -> Hook_rear/15  "Local_force_Z"
  Demux/237 -> Hook_rear/14  "Local_force_Y"
  Demux/236 -> Hook_rear/13  "Local_force_X"
  Demux/235 -> Hook_rear/12  "Hook_Z"
  Demux/234 -> Hook_rear/11  "Hook_Y"
  Demux/233 -> Hook_rear/10  "Hook_X"
  Demux/232 -> Hook_rear/9  "Hook_Theta"
  Demux/231 -> Hook_rear/8  "Hook_Psi"
  Demux/230 -> Hook_rear/7  "Hook_Phi"
  Demux/229 -> Hook_rear/6  "Global_Moment_Z"
  Demux/228 -> Hook_rear/5  "Global_Moment_Y"
  Demux/227 -> Hook_rear/4  "Global_Moment_X"
  Demux/226 -> Hook_rear/3  "Global_force_Z"
  Demux/225 -> Hook_rear/2  "Global_force_Y"
  Demux/224 -> Hook_rear/1  "Global_force_X"
  Hook_rear/1 -> OutputBus/31  "Hook_rear"
  Demux/223 -> Gyro/10  "sensor_3_Z"
  Demux/222 -> Gyro/9  "sensor_2_Z"
  Demux/221 -> Gyro/8  "sensor_1_Z"
  Demux/220 -> Gyro/7  "gyro_Y"
  Demux/219 -> Gyro/6  "gyro_X"
  Demux/218 -> Gyro/5  "gyro_VX"
  Demux/217 -> Gyro/4  "gyro_ACCY"
  Demux/216 -> Gyro/3  "gyro_ACCX"
  Demux/215 -> Gyro/2  "Driver_Z"
  Demux/214 -> Gyro/1  "Driver_X"
  Gyro/1 -> OutputBus/30  "Gyro"
  Demux/213 -> ges_chassis_XFORM/6  "Z"
  Demux/212 -> ges_chassis_XFORM/5  "Y"
  Demux/211 -> ges_chassis_XFORM/4  "X"
  Demux/210 -> ges_chassis_XFORM/3  "Theta"
  Demux/209 -> ges_chassis_XFORM/2  "Psi"
  Demux/208 -> ges_chassis_XFORM/1  "Phi"
  ges_chassis_XFORM/1 -> OutputBus/29  "ges_chassis_XFORM"
  Demux/207 -> fuel_consumption/4  "overall"
  Demux/206 -> fuel_consumption/3  "instantaneous_Liter_100km"
  Demux/205 -> fuel_consumption/2  "instantaneous"
  Demux/204 -> fuel_consumption/1  "BSFC"
  fuel_consumption/1 -> OutputBus/28  "fuel_consumption"
  Demux/203 -> engine/7  "torque"
  Demux/202 -> engine/6  "Power_KW"
  Demux/201 -> engine/5  "Power_HP"
  Demux/200 -> engine/4  "Min_engine_torque"
  Demux/199 -> engine/3  "Max_Engine_torque"
  Demux/198 -> engine/2  "engine_rpm"
  Demux/197 -> engine/1  "effective_throttle"
  engine/1 -> OutputBus/27  "engine"
  Demux/196 -> driving_machine_monitor/9  "target_vx"
  Demux/195 -> driving_machine_monitor/8  "target_ax"
  Demux/194 -> driving_machine_monitor/7  "path_z"
  Demux/193 -> driving_machine_monitor/6  "path_y"
  Demux/192 -> driving_machine_monitor/5  "path_x"
  Demux/191 -> driving_machine_monitor/4  "path_s"
  Demux/190 -> driving_machine_monitor/3  "path_distance"
  Demux/189 -> driving_machine_monitor/2  "path_curvature"
  Demux/188 -> driving_machine_monitor/1  "maneuver_ID"
  driving_machine_monitor/1 -> OutputBus/26  "driving_machine_monitor"
  Demux/187 -> driver_demands/7  "throttle"
  Demux/186 -> driver_demands/6  "steering_velocity"
  Demux/185 -> driver_demands/5  "steering"
  Demux/184 -> driver_demands/4  "gear"
  Demux/183 -> driver_demands/3  "clutch"
  Demux/182 -> driver_demands/2  "brake_pressure"
  Demux/181 -> driver_demands/1  "brake"
  driver_demands/1 -> OutputBus/25  "driver_demands"
  Demux/180 -> differential_torques/6  "output_torque_right_rear"
  Demux/179 -> differential_torques/5  "output_torque_right_front"
  Demux/178 -> differential_torques/4  "output_torque_left_rear"
  Demux/177 -> differential_torques/3  "output_torque_left_front"
  Demux/176 -> differential_torques/2  "differential_torque_rear"
  Demux/175 -> differential_torques/1  "differential_torque_front"
  differential_torques/1 -> OutputBus/24  "differential_torques"
  Demux/174 -> differential_speeds/6  "halfshaft_omega_right_rear"
  Demux/173 -> differential_speeds/5  "halfshaft_omega_right_front"
  Demux/172 -> differential_speeds/4  "halfshaft_omega_left_rear"
  Demux/171 -> differential_speeds/3  "halfshaft_omega_left_front"
  Demux/170 -> differential_speeds/2  "halfshaft_omega_delta_rear"
  Demux/169 -> differential_speeds/1  "halfshaft_omega_delta_front"
  differential_speeds/1 -> OutputBus/23  "differential_speeds"
  Demux/168 -> das_third_damper_data/6  "velocity_rear"
  Demux/167 -> das_third_damper_data/5  "velocity_front"
  Demux/166 -> das_third_damper_data/4  "force_rear"
  Demux/165 -> das_third_damper_data/3  "force_front"
  Demux/164 -> das_third_damper_data/2  "displacement_rear"
  Demux/163 -> das_third_damper_data/1  "displacement_front"
  das_third_damper_data/1 -> OutputBus/22  "das_third_damper_data"
  Demux/162 -> das_roll_damper_data/8  "velocity_rear"
  Demux/161 -> das_roll_damper_data/7  "velocity_front"
  Demux/160 -> das_roll_damper_data/6  "force_rear"
  Demux/159 -> das_roll_damper_data/5  "force_front"
  Demux/158 -> das_roll_damper_data/4  "force_at_wheel_rear"
  Demux/157 -> das_roll_damper_data/3  "force_at_wheel_front"
  Demux/156 -> das_roll_damper_data/2  "displacement_rear"
  Demux/155 -> das_roll_damper_data/1  "displacement_front"
  das_roll_damper_data/1 -> OutputBus/21  "das_roll_damper_data"
  Demux/154 -> das_ride_damper_data/6  "velocity_rear"
  Demux/153 -> das_ride_damper_data/5  "velocity_front"
  Demux/152 -> das_ride_damper_data/4  "force_rear"
  Demux/151 -> das_ride_damper_data/3  "force_front"
  Demux/150 -> das_ride_damper_data/2  "displacement_rear"
  Demux/149 -> das_ride_damper_data/1  "displacement_front"
  das_ride_damper_data/1 -> OutputBus/20  "das_ride_damper_data"
  Demux/148 -> dar_ride_damper_data/4  "velocity_rear"
  Demux/147 -> dar_ride_damper_data/3  "velocity_front"
  Demux/146 -> dar_ride_damper_data/2  "force_rear"
  Demux/145 -> dar_ride_damper_data/1  "force_front"
  dar_ride_damper_data/1 -> OutputBus/19  "dar_ride_damper_data"
  Demux/144 -> Jounce_Rate/4  "R2"
  Demux/143 -> Jounce_Rate/3  "R1"
  Demux/142 -> Jounce_Rate/2  "L2"
  Demux/141 -> Jounce_Rate/1  "L1"
  Jounce_Rate/1 -> Damper/5  "Jounce_Rate"
  Demux/140 -> Jounce_Acceleration/4  "R2"
  Demux/139 -> Jounce_Acceleration/3  "R1"
  Demux/138 -> Jounce_Acceleration/2  "L2"
  Demux/137 -> Jounce_Acceleration/1  "L1"
  Jounce_Acceleration/1 -> Damper/4  "Jounce_Acceleration"
  Demux/136 -> Jounce/4  "R2"
  Demux/135 -> Jounce/3  "R1"
  Demux/134 -> Jounce/2  "L2"
  Demux/133 -> Jounce/1  "L1"
  Jounce/1 -> Damper/3  "Jounce"
  Demux/132 -> Force_At_Wheel/4  "R2"
  Demux/131 -> Force_At_Wheel/3  "R1"
  Demux/130 -> Force_At_Wheel/2  "L2"
  Demux/129 -> Force_At_Wheel/1  "L1"
  Force_At_Wheel/1 -> Damper/2  "Force_At_Wheel"
  Demux/128 -> Force_At_Damper/4  "R2"
  Demux/127 -> Force_At_Damper/3  "R1"
  Demux/126 -> Force_At_Damper/2  "L2"
  Demux/125 -> Force_At_Damper/1  "L1"
  Force_At_Damper/1 -> Damper/1  "Force_At_Damper"
  Damper/1 -> OutputBus/18  "Damper"
  Demux/124 -> dal_ride_damper_data/4  "velocity_rear"
  Demux/123 -> dal_ride_damper_data/3  "velocity_front"
  Demux/122 -> dal_ride_damper_data/2  "force_rear"
  Demux/121 -> dal_ride_damper_data/1  "force_front"
  dal_ride_damper_data/1 -> OutputBus/17  "dal_ride_damper_data"
  Demux/120 -> cross_weight/4  "side_right_ratio"
  Demux/119 -> cross_weight/3  "nose_ratio"
  Demux/118 -> cross_weight/2  "crossR1L2_ratio"
  Demux/117 -> cross_weight/1  "crossL1R2_ratio"
  cross_weight/1 -> OutputBus/16  "cross_weight"
  Demux/116 -> condition_sensors/1  "side_slip_angle"
  condition_sensors/1 -> OutputBus/15  "condition_sensors"
  Demux/115 -> clutch/2  "torque"
  Demux/114 -> clutch/1  "slip_angle"
  clutch/1 -> OutputBus/14  "clutch"
  Demux/113 -> chassis_velocities/6  "yaw"
  Demux/112 -> chassis_velocities/5  "vertical"
  Demux/111 -> chassis_velocities/4  "roll"
  Demux/110 -> chassis_velocities/3  "pitch"
  Demux/109 -> chassis_velocities/2  "longitudinal"
  Demux/108 -> chassis_velocities/1  "lateral"
  chassis_velocities/1 -> OutputBus/13  "chassis_velocities"
  Demux/107 -> chassis_displacements/9  "yaw"
  Demux/106 -> chassis_displacements/8  "vertical_wrt_road"
  Demux/105 -> chassis_displacements/7  "vertical"
  Demux/104 -> chassis_displacements/6  "roll_wrt_road"
  Demux/103 -> chassis_displacements/5  "roll"
  Demux/102 -> chassis_displacements/4  "pitch_wrt_road"
  Demux/101 -> chassis_displacements/3  "pitch"
  Demux/100 -> chassis_displacements/2  "longitudinal"
  Demux/99 -> chassis_displacements/1  "lateral"
  chassis_displacements/1 -> OutputBus/12  "chassis_displacements"
  Demux/98 -> chassis_accelerations/6  "yaw"
  Demux/97 -> chassis_accelerations/5  "vertical"
  Demux/96 -> chassis_accelerations/4  "roll"
  Demux/95 -> chassis_accelerations/3  "pitch"
  Demux/94 -> chassis_accelerations/2  "longitudinal"
  Demux/93 -> chassis_accelerations/1  "lateral"
  chassis_accelerations/1 -> OutputBus/11  "chassis_accelerations"
  Demux/92 -> bus_spr_jounce_stop_data/6  "velocity_rear"
  Demux/91 -> bus_spr_jounce_stop_data/5  "velocity_front"
  Demux/90 -> bus_spr_jounce_stop_data/4  "force_rear"
  Demux/89 -> bus_spr_jounce_stop_data/3  "force_front"
  Demux/88 -> bus_spr_jounce_stop_data/2  "displacement_rear"
  Demux/87 -> bus_spr_jounce_stop_data/1  "displacement_front"
  bus_spr_jounce_stop_data/1 -> OutputBus/10  "bus_spr_jounce_stop_data"
  Demux/86 -> bus_roll_dmp_jounce_stop_data/6  "velocity_rear"
  Demux/85 -> bus_roll_dmp_jounce_stop_data/5  "velocity_front"
  Demux/84 -> bus_roll_dmp_jounce_stop_data/4  "force_rear"
  Demux/83 -> bus_roll_dmp_jounce_stop_data/3  "force_front"
  Demux/82 -> bus_roll_dmp_jounce_stop_data/2  "displacement_rear"
  Demux/81 -> bus_roll_dmp_jounce_stop_data/1  "displacement_front"
  bus_roll_dmp_jounce_stop_data/1 -> OutputBus/9  "bus_roll_dmp_jounce_stop_data"
  Demux/80 -> bus_ins_jounce_stop_data/6  "velocity_rear"
  Demux/79 -> bus_ins_jounce_stop_data/5  "velocity_front"
  Demux/78 -> bus_ins_jounce_stop_data/4  "force_rear"
  Demux/77 -> bus_ins_jounce_stop_data/3  "force_front"
  Demux/76 -> bus_ins_jounce_stop_data/2  "displacement_rear"
  Demux/75 -> bus_ins_jounce_stop_data/1  "displacement_front"
  bus_ins_jounce_stop_data/1 -> OutputBus/8  "bus_ins_jounce_stop_data"
  Demux/74 -> bus_dmp_jounce_stop_data/6  "velocity_rear"
  Demux/73 -> bus_dmp_jounce_stop_data/5  "velocity_front"
  Demux/72 -> bus_dmp_jounce_stop_data/4  "force_rear"
  Demux/71 -> bus_dmp_jounce_stop_data/3  "force_front"
  Demux/70 -> bus_dmp_jounce_stop_data/2  "displacement_rear"
  Demux/69 -> bus_dmp_jounce_stop_data/1  "displacement_front"
  bus_dmp_jounce_stop_data/1 -> OutputBus/7  "bus_dmp_jounce_stop_data"
  Demux/68 -> bur_rebound_stop_data/4  "velocity_rear"
  Demux/67 -> bur_rebound_stop_data/3  "velocity_front"
  Demux/66 -> bur_rebound_stop_data/2  "force_rear"
  Demux/65 -> bur_rebound_stop_data/1  "force_front"
  bur_rebound_stop_data/1 -> OutputBus/6  "bur_rebound_stop_data"
  Demux/64 -> bur_jounce_stop_data/4  "velocity_rear"
  Demux/63 -> bur_jounce_stop_data/3  "velocity_front"
  Demux/62 -> bur_jounce_stop_data/2  "force_rear"
  Demux/61 -> bur_jounce_stop_data/1  "force_front"
  bur_jounce_stop_data/1 -> OutputBus/5  "bur_jounce_stop_data"
  Demux/60 -> bul_rebound_stop_data/4  "velocity_rear"
  Demux/59 -> bul_rebound_stop_data/3  "velocity_front"
  Demux/58 -> bul_rebound_stop_data/2  "force_rear"
  Demux/57 -> bul_rebound_stop_data/1  "force_front"
  bul_rebound_stop_data/1 -> OutputBus/4  "bul_rebound_stop_data"
  Demux/56 -> bul_jounce_stop_data/4  "velocity_rear"
  Demux/55 -> bul_jounce_stop_data/3  "velocity_front"
  Demux/54 -> bul_jounce_stop_data/2  "force_rear"
  Demux/53 -> bul_jounce_stop_data/1  "force_front"
  bul_jounce_stop_data/1 -> OutputBus/3  "bul_jounce_stop_data"
  Demux/52 -> Lockup_Rotation/4  "R2"
  Demux/51 -> Lockup_Rotation/3  "R1"
  Demux/50 -> Lockup_Rotation/2  "L2"
  Demux/49 -> Lockup_Rotation/1  "L1"
  Lockup_Rotation/1 -> Brake/7  "Lockup_Rotation"
  Demux/48 -> Locked_Switch/4  "R2"
  Demux/47 -> Locked_Switch/3  "R1"
  Demux/46 -> Locked_Switch/2  "L2"
  Demux/45 -> Locked_Switch/1  "L1"
  Locked_Switch/1 -> Brake/6  "Locked_Switch"
  Demux/44 -> Locked_Spring_Moment/4  "R2"
  Demux/43 -> Locked_Spring_Moment/3  "R1"
  Demux/42 -> Locked_Spring_Moment/2  "L2"
  Demux/41 -> Locked_Spring_Moment/1  "L1"
  Locked_Spring_Moment/1 -> Brake/5  "Locked_Spring_Moment"
  Demux/40 -> Locked_Moment/4  "R2"
  Demux/39 -> Locked_Moment/3  "R1"
  Demux/38 -> Locked_Moment/2  "L2"
  Demux/37 -> Locked_Moment/1  "L1"
  Locked_Moment/1 -> Brake/4  "Locked_Moment"
  Demux/36 -> Locked_Damper_Moment/4  "R2"
  Demux/35 -> Locked_Damper_Moment/3  "R1"
  Demux/34 -> Locked_Damper_Moment/2  "L2"
  Demux/33 -> Locked_Damper_Moment/1  "L1"
  Locked_Damper_Moment/1 -> Brake/3  "Locked_Damper_Moment"
  Demux/32 -> Chamber_Pressure/4  "R2"
  Demux/31 -> Chamber_Pressure/3  "R1"
  Demux/30 -> Chamber_Pressure/2  "L2"
  Demux/29 -> Chamber_Pressure/1  "L1"
  Chamber_Pressure/1 -> Brake/2  "Chamber_Pressure"
  Demux/28 -> Brake_Moment/4  "R2"
  Demux/27 -> Brake_Moment/3  "R1"
  Demux/26 -> Brake_Moment/2  "L2"
  Demux/25 -> Brake_Moment/1  "L1"
  Brake_Moment/1 -> Brake/1  "Brake_Moment"
  Brake/1 -> OutputBus/2  "Brake"
  Demux/24 -> aero_forces/24  "yaw_torque"
  Demux/23 -> aero_forces/23  "vertical_velocity"
  Demux/22 -> aero_forces/22  "steer"
  Demux/21 -> aero_forces/21  "side_slip"
  Demux/20 -> aero_forces/20  "roll_torque"
  Demux/19 -> aero_forces/19  "roll"
  Demux/18 -> aero_forces/18  "rear_sideforce"
  Demux/17 -> aero_forces/17  "rear_downforce"
  Demux/16 -> aero_forces/16  "pitch"
  Demux/15 -> aero_forces/15  "longitudinal_velocity"
  Demux/14 -> aero_forces/14  "lateral_velocity"
  Demux/13 -> aero_forces/13  "height_rear"
  Demux/12 -> aero_forces/12  "height_front"
  Demux/11 -> aero_forces/11  "height_auxiliary"
  Demux/10 -> aero_forces/10  "front_sideforce"
  Demux/9 -> aero_forces/9  "front_downforce"
  Demux/8 -> aero_forces/8  "drag_torque"
  Demux/7 -> aero_forces/7  "drag_force_rear"
  Demux/6 -> aero_forces/6  "drag_force_front"
  Demux/5 -> aero_forces/5  "drag_force"
  Demux/4 -> aero_forces/4  "drag_arm"
  Demux/3 -> aero_forces/3  "center_sideforce"
  Demux/2 -> aero_forces/2  "center_downforce"
  Demux/1 -> aero_forces/1  "aero_balance"
  aero_forces/1 -> OutputBus/1  "aero_forces"
  OutputBus/1 -> Out/1  "OutputBus"
  In/1 -> Demux/1
